simulink library "outp"  (R2021b)
(part 8 of 10)

      link override Signal_Override/_ovrdflg: Value=KOUTP_EC1EMSupVarRTSC1MSG_cnt_ovrdflg
      link override Signal_Override/_ovrdval: Value=KOUTP_EC1EMSupVarRTSC1MSG_cnt_ovrdval
  VTQD_EC1PercTorqIdleP1_pct_Inproc : FVT_lib/outp/OverrideAndLimit  SystemSampleTime=-1  VariantActivationTime=update diagram  Latency=0  AutoFrameSizeCalculation=off
      link override Signal_Limit/_maxval: Value=KOUTP_EC1PercTorqIdleP1_pct_maxval
      link override Signal_Limit/_minval: Value=KOUTP_EC1PercTorqIdleP1_pct_minval
      link override Signal_Override/_ovrdflg: Value=KOUTP_EC1PercTorqIdleP1_pct_ovrdflg
      link override Signal_Override/_ovrdval: Value=KOUTP_EC1PercTorqIdleP1_pct_ovrdval
  VTQD_EC1PercTorqIdleP2_pct_Inproc : FVT_lib/outp/OverrideAndLimit  SystemSampleTime=-1  VariantActivationTime=update diagram  Latency=0  AutoFrameSizeCalculation=off
      link override Signal_Limit/_maxval: Value=KOUTP_EC1PercTorqIdleP2_pct_maxval
      link override Signal_Limit/_minval: Value=KOUTP_EC1PercTorqIdleP2_pct_minval
      link override Signal_Override/_ovrdflg: Value=KOUTP_EC1PercTorqIdleP2_pct_ovrdflg
      link override Signal_Override/_ovrdval: Value=KOUTP_EC1PercTorqIdleP2_pct_ovrdval
  VTQD_EC1PercTorqIdleP3_pct_Inproc : FVT_lib/outp/OverrideAndLimit  SystemSampleTime=-1  VariantActivationTime=update diagram  Latency=0  AutoFrameSizeCalculation=off
      link override Signal_Limit/_maxval: Value=KOUTP_EC1PercTorqIdleP3_pct_maxval
      link override Signal_Limit/_minval: Value=KOUTP_EC1PercTorqIdleP3_pct_minval
      link override Signal_Override/_ovrdflg: Value=KOUTP_EC1PercTorqIdleP3_pct_ovrdflg
      link override Signal_Override/_ovrdval: Value=KOUTP_EC1PercTorqIdleP3_pct_ovrdval
  VTQD_EC1PercTorqIdleP4_pct_Inproc : FVT_lib/outp/OverrideAndLimit  SystemSampleTime=-1  VariantActivationTime=update diagram  Latency=0  AutoFrameSizeCalculation=off
      link override Signal_Limit/_maxval: Value=KOUTP_EC1PercTorqIdleP4_pct_maxval
      link override Signal_Limit/_minval: Value=KOUTP_EC1PercTorqIdleP4_pct_minval
      link override Signal_Override/_ovrdflg: Value=KOUTP_EC1PercTorqIdleP4_pct_ovrdflg
      link override Signal_Override/_ovrdval: Value=KOUTP_EC1PercTorqIdleP4_pct_ovrdval
  VTQD_EC1PercTorqIdleP5_pct_Inproc : FVT_lib/outp/OverrideAndLimit  SystemSampleTime=-1  VariantActivationTime=update diagram  Latency=0  AutoFrameSizeCalculation=off
      link override Signal_Limit/_maxval: Value=KOUTP_EC1PercTorqIdleP5_pct_maxval
      link override Signal_Limit/_minval: Value=KOUTP_EC1PercTorqIdleP5_pct_minval
      link override Signal_Override/_ovrdflg: Value=KOUTP_EC1PercTorqIdleP5_pct_ovrdflg
      link override Signal_Override/_ovrdval: Value=KOUTP_EC1PercTorqIdleP5_pct_ovrdval
  VTQD_EEC3EMPressLoss_pct_Inproc : FVT_lib/outp/OverrideAndLimit  SystemSampleTime=-1  VariantActivationTime=update diagram  Latency=0  AutoFrameSizeCalculation=off
      link override Signal_Limit/_maxval: Value=KOUTP_EEC3EMPressLoss_pct_maxval
      link override Signal_Limit/_minval: Value=KOUTP_EEC3EMPressLoss_pct_minval
      link override Signal_Override/_ovrdflg: Value=KOUTP_EEC3EMPressLoss_pct_ovrdflg
      link override Signal_Override/_ovrdval: Value=KOUTP_EEC3EMPressLoss_pct_ovrdval
  VTQD_EEC3NFricPercTorq_pct_Inproc : FVT_lib/outp/OverrideAndLimit  SystemSampleTime=-1  VariantActivationTime=update diagram  Latency=0  AutoFrameSizeCalculation=off
      link override Signal_Limit/_maxval: Value=KOUTP_EEC3NFricPercTorq_pct_maxval
      link override Signal_Limit/_minval: Value=KOUTP_EEC3NFricPercTorq_pct_minval
      link override Signal_Override/_ovrdflg: Value=KOUTP_EEC3NFricPercTorq_pct_ovrdflg
      link override Signal_Override/_ovrdval: Value=KOUTP_EEC3NFricPercTorq_pct_ovrdval
  VTQD_EMRC1ActEMOutSftSpd_rpm_Inproc : FVT_lib/outp/OverrideAndLimit  SystemSampleTime=-1  VariantActivationTime=update diagram  Latency=0  AutoFrameSizeCalculation=off
      link override Signal_Limit/_maxval: Value=KOUTP_EMRC1ActEMOutSftSpd_rpm_maxval
      link override Signal_Limit/_minval: Value=KOUTP_EMRC1ActEMOutSftSpd_rpm_minval
      link override Signal_Override/_ovrdflg: Value=KOUTP_EMRC1ActEMOutSftSpd_rpm_ovrdflg
      link override Signal_Override/_ovrdval: Value=KOUTP_EMRC1ActEMOutSftSpd_rpm_ovrdval
  VTQD_EMRC1ActEMpTrqHrls_pct_Inproc : FVT_lib/outp/OverrideAndLimit  SystemSampleTime=-1  VariantActivationTime=update diagram  Latency=0  AutoFrameSizeCalculation=off
      link override Signal_Limit/_maxval: Value=KOUTP_EMRC1ActEMpTrqHrls_pct_maxval
      link override Signal_Limit/_minval: Value=KOUTP_EMRC1ActEMpTrqHrls_pct_minval
      link override Signal_Override/_ovrdflg: Value=KOUTP_EMRC1ActEMpTrqHrls_pct_ovrdflg
      link override Signal_Override/_ovrdval: Value=KOUTP_EMRC1ActEMpTrqHrls_pct_ovrdval
  VTQD_EMRC1ActEMpTrq_pct_Inproc : FVT_lib/outp/OverrideAndLimit  SystemSampleTime=-1  VariantActivationTime=update diagram  Latency=0  AutoFrameSizeCalculation=off
      link override Signal_Limit/_maxval: Value=KOUTP_EMRC1ActEMpTrq_pct_maxval
      link override Signal_Limit/_minval: Value=KOUTP_EMRC1ActEMpTrq_pct_minval
      link override Signal_Override/_ovrdflg: Value=KOUTP_EMRC1ActEMpTrq_pct_ovrdflg
      link override Signal_Override/_ovrdval: Value=KOUTP_EMRC1ActEMpTrq_pct_ovrdval
  VTQD_EMRC1ActMaxAvaEMRecpTrq_pct_Inproc : FVT_lib/outp/OverrideAndLimit  SystemSampleTime=-1  VariantActivationTime=update diagram  Latency=0  AutoFrameSizeCalculation=off
      link override Signal_Limit/_maxval: Value=KOUTP_EMRC1ActMaxAvaEMRecpTrq_pct_maxval
      link override Signal_Limit/_minval: Value=KOUTP_EMRC1ActMaxAvaEMRecpTrq_pct_minval
      link override Signal_Override/_ovrdflg: Value=KOUTP_EMRC1ActMaxAvaEMRecpTrq_pct_ovrdflg
      link override Signal_Override/_ovrdval: Value=KOUTP_EMRC1ActMaxAvaEMRecpTrq_pct_ovrdval
  VTQD_EMRC1DrvDemEMRtapTrq_pct_Inproc : FVT_lib/outp/OverrideAndLimit  SystemSampleTime=-1  VariantActivationTime=update diagram  Latency=0  AutoFrameSizeCalculation=off
      link override Signal_Limit/_maxval: Value=KOUTP_EMRC1DrvDemEMRtapTrq_pct_maxval
      link override Signal_Limit/_minval: Value=KOUTP_EMRC1DrvDemEMRtapTrq_pct_minval
      link override Signal_Override/_ovrdflg: Value=KOUTP_EMRC1DrvDemEMRtapTrq_pct_ovrdflg
      link override Signal_Override/_ovrdval: Value=KOUTP_EMRC1DrvDemEMRtapTrq_pct_ovrdval
  VTQD_EMRC1EMTquModeDrvBrk_enum_Inproc : FVT_lib/outp/OverrideAndLimit  SystemSampleTime=-1  VariantActivationTime=update diagram  Latency=0  AutoFrameSizeCalculation=off
      link override Signal_Limit/_maxval: Value=KOUTP_EMRC1EMTquModeDrvBrk_enum_maxval
      link override Signal_Limit/_minval: Value=KOUTP_EMRC1EMTquModeDrvBrk_enum_minval
      link override Signal_Override/_ovrdflg: Value=KOUTP_EMRC1EMTquModeDrvBrk_enum_ovrdflg
      link override Signal_Override/_ovrdval: Value=KOUTP_EMRC1EMTquModeDrvBrk_enum_ovrdval
  VTQD_EMRC1RetSelNonEng_pct_Inproc : FVT_lib/outp/OverrideAndLimit  SystemSampleTime=-1  VariantActivationTime=update diagram  Latency=0  AutoFrameSizeCalculation=off
      link override Signal_Limit/_maxval: Value=KOUTP_EMRC1RetSelNonEng_pct_maxval
      link override Signal_Limit/_minval: Value=KOUTP_EMRC1RetSelNonEng_pct_minval
      link override Signal_Override/_ovrdflg: Value=KOUTP_EMRC1RetSelNonEng_pct_ovrdflg
      link override Signal_Override/_ovrdval: Value=KOUTP_EMRC1RetSelNonEng_pct_ovrdval
  VTQD_EMRC1SACtrlDev_cnt_Inproc : FVT_lib/outp/OverrideAndLimit  SystemSampleTime=-1  VariantActivationTime=update diagram  Latency=0  AutoFrameSizeCalculation=off
      link override Signal_Limit/_maxval: Value=KOUTP_EMRC1SACtrlDev_cnt_maxval
      link override Signal_Limit/_minval: Value=KOUTP_EMRC1SACtrlDev_cnt_minval
      link override Signal_Override/_ovrdflg: Value=KOUTP_EMRC1SACtrlDev_cnt_ovrdflg
      link override Signal_Override/_ovrdval: Value=KOUTP_EMRC1SACtrlDev_cnt_ovrdval
  VTQD_ETC1ShiftrPgs_enum_Inproc : FVT_lib/outp/OverrideAndLimit  SystemSampleTime=-1  VariantActivationTime=update diagram  Latency=0  AutoFrameSizeCalculation=off
      link override Signal_Limit/_maxval: Value=KOUTP_ETC1ShiftrPgs_enum_maxval
      link override Signal_Limit/_minval: Value=KOUTP_ETC1ShiftrPgs_enum_minval
      link override Signal_Override/_ovrdflg: Value=KOUTP_ETC1ShiftrPgs_enum_ovrdflg
      link override Signal_Override/_ovrdval: Value=KOUTP_ETC1ShiftrPgs_enum_ovrdval
  VTQD_ETC2ActDriveDirect_enum_Inproc : FVT_lib/outp/OverrideAndLimit  SystemSampleTime=-1  VariantActivationTime=update diagram  Latency=0  AutoFrameSizeCalculation=off
      link override Signal_Limit/_maxval: Value=KOUTP_ETC2ActDriveDirect_enum_maxval
      link override Signal_Limit/_minval: Value=KOUTP_ETC2ActDriveDirect_enum_minval
      link override Signal_Override/_ovrdflg: Value=KOUTP_ETC2ActDriveDirect_enum_ovrdflg
      link override Signal_Override/_ovrdval: Value=KOUTP_ETC2ActDriveDirect_enum_ovrdval
  VTQD_EVCU1ActDrvMode_enum_Inproc : FVT_lib/outp/OverrideAndLimit  SystemSampleTime=-1  VariantActivationTime=update diagram  Latency=0  AutoFrameSizeCalculation=off
      link override Signal_Limit/_maxval: Value=KOUTP_EVCU1ActDrvMode_enum_maxval
      link override Signal_Limit/_minval: Value=KOUTP_EVCU1ActDrvMode_enum_minval
      link override Signal_Override/_ovrdflg: Value=KOUTP_EVCU1ActDrvMode_enum_ovrdflg
      link override Signal_Override/_ovrdval: Value=KOUTP_EVCU1ActDrvMode_enum_ovrdval
  VTQD_EVCU1EBrakeTorqLow_enum_Inproc : FVT_lib/outp/OverrideAndLimit  SystemSampleTime=-1  VariantActivationTime=update diagram  Latency=0  AutoFrameSizeCalculation=off
      link override Signal_Limit/_maxval: Value=KOUTP_EVCU1EBrakeTorqLow_enum_maxval
      link override Signal_Limit/_minval: Value=KOUTP_EVCU1EBrakeTorqLow_enum_minval
      link override Signal_Override/_ovrdflg: Value=KOUTP_EVCU1EBrakeTorqLow_enum_ovrdflg
      link override Signal_Override/_ovrdval: Value=KOUTP_EVCU1EBrakeTorqLow_enum_ovrdval
  VTQD_EVCU1EMotorOvrerSpd_enum_Inproc : FVT_lib/outp/OverrideAndLimit  SystemSampleTime=-1  VariantActivationTime=update diagram  Latency=0  AutoFrameSizeCalculation=off
      link override Signal_Limit/_maxval: Value=KOUTP_EVCU1EMotorOvrerSpd_enum_maxval
      link override Signal_Limit/_minval: Value=KOUTP_EVCU1EMotorOvrerSpd_enum_minval
      link override Signal_Override/_ovrdflg: Value=KOUTP_EVCU1EMotorOvrerSpd_enum_ovrdflg
      link override Signal_Override/_ovrdval: Value=KOUTP_EVCU1EMotorOvrerSpd_enum_ovrdval
  VTQD_EVCU1EMotorPerformance_pct_Inproc : FVT_lib/outp/OverrideAndLimit  SystemSampleTime=-1  VariantActivationTime=update diagram  Latency=0  AutoFrameSizeCalculation=off
      link override Signal_Limit/_maxval: Value=KOUTP_EVCU1EMotorPerformance_pct_maxval
      link override Signal_Limit/_minval: Value=KOUTP_EVCU1EMotorPerformance_pct_minval
      link override Signal_Override/_ovrdflg: Value=KOUTP_EVCU1EMotorPerformance_pct_ovrdflg
      link override Signal_Override/_ovrdval: Value=KOUTP_EVCU1EMotorPerformance_pct_ovrdval
  VTQD_EVCU1EMotorSpd_rpm_Inproc : FVT_lib/outp/OverrideAndLimit  SystemSampleTime=-1  VariantActivationTime=update diagram  Latency=0  AutoFrameSizeCalculation=off
      link override Signal_Limit/_maxval: Value=KOUTP_EVCU1EMotorSpd_rpm_maxval
      link override Signal_Limit/_minval: Value=KOUTP_EVCU1EMotorSpd_rpm_minval
      link override Signal_Override/_ovrdflg: Value=KOUTP_EVCU1EMotorSpd_rpm_ovrdflg
      link override Signal_Override/_ovrdval: Value=KOUTP_EVCU1EMotorSpd_rpm_ovrdval
  VTQD_EVCU1RecuperHighSta_enum_Inproc : FVT_lib/outp/OverrideAndLimit  SystemSampleTime=-1  VariantActivationTime=update diagram  Latency=0  AutoFrameSizeCalculation=off
      link override Signal_Limit/_maxval: Value=KOUTP_EVCU1RecuperHighSta_enum_maxval
      link override Signal_Limit/_minval: Value=KOUTP_EVCU1RecuperHighSta_enum_minval
      link override Signal_Override/_ovrdflg: Value=KOUTP_EVCU1RecuperHighSta_enum_ovrdflg
      link override Signal_Override/_ovrdval: Value=KOUTP_EVCU1RecuperHighSta_enum_ovrdval
  VTQD_EVCU1WheelSlipdet_enum_Inproc : FVT_lib/outp/OverrideAndLimit  SystemSampleTime=-1  VariantActivationTime=update diagram  Latency=0  AutoFrameSizeCalculation=off
      link override Signal_Limit/_maxval: Value=KOUTP_EVCU1WheelSlipdet_enum_maxval
      link override Signal_Limit/_minval: Value=KOUTP_EVCU1WheelSlipdet_enum_minval
      link override Signal_Override/_ovrdflg: Value=KOUTP_EVCU1WheelSlipdet_enum_ovrdflg
      link override Signal_Override/_ovrdval: Value=KOUTP_EVCU1WheelSlipdet_enum_ovrdval
  VTQD_EVCU2MaxTorqAvail_pct_Inproc : FVT_lib/outp/OverrideAndLimit  SystemSampleTime=-1  VariantActivationTime=update diagram  Latency=0  AutoFrameSizeCalculation=off
      link override Signal_Limit/_maxval: Value=KOUTP_EVCU2MaxTorqAvail_pct_maxval
      link override Signal_Limit/_minval: Value=KOUTP_EVCU2MaxTorqAvail_pct_minval
      link override Signal_Override/_ovrdflg: Value=KOUTP_EVCU2MaxTorqAvail_pct_ovrdflg
      link override Signal_Override/_ovrdval: Value=KOUTP_EVCU2MaxTorqAvail_pct_ovrdval
  VTQD_EVCU2MinTorqAvail_pct_Inproc : FVT_lib/outp/OverrideAndLimit  SystemSampleTime=-1  VariantActivationTime=update diagram  Latency=0  AutoFrameSizeCalculation=off
      link override Signal_Limit/_maxval: Value=KOUTP_EVCU2MinTorqAvail_pct_maxval
      link override Signal_Limit/_minval: Value=KOUTP_EVCU2MinTorqAvail_pct_minval
      link override Signal_Override/_ovrdflg: Value=KOUTP_EVCU2MinTorqAvail_pct_ovrdflg
      link override Signal_Override/_ovrdval: Value=KOUTP_EVCU2MinTorqAvail_pct_ovrdval
  VTQD_GearFlashIndDis_flg_Inproc : FVT_lib/outp/OverrideAndLimit  SystemSampleTime=-1  VariantActivationTime=update diagram  Latency=0  AutoFrameSizeCalculation=off
      link override Signal_Limit/_maxval: Value=KOUTP_GearFlashIndDis_flg_maxval
      link override Signal_Limit/_minval: Value=KOUTP_GearFlashIndDis_flg_minval
      link override Signal_Override/_ovrdflg: Value=KOUTP_GearFlashIndDis_flg_ovrdflg
      link override Signal_Override/_ovrdval: Value=KOUTP_GearFlashIndDis_flg_ovrdval
  VTQD_GearFlashInd_flg_Inproc : FVT_lib/outp/OverrideAndLimit  SystemSampleTime=-1  VariantActivationTime=update diagram  Latency=0  AutoFrameSizeCalculation=off
      link override Signal_Limit/_maxval: Value=KOUTP_GearFlashInd_flg_maxval
      link override Signal_Limit/_minval: Value=KOUTP_GearFlashInd_flg_minval
      link override Signal_Override/_ovrdflg: Value=KOUTP_GearFlashInd_flg_ovrdflg
      link override Signal_Override/_ovrdval: Value=KOUTP_GearFlashInd_flg_ovrdval
  VTQD_ParkingProtectWarning_flg_Inproc : FVT_lib/outp/OverrideAndLimit  SystemSampleTime=-1  VariantActivationTime=update diagram  Latency=0  AutoFrameSizeCalculation=off
      link override Signal_Limit/_maxval: Value=KOUTP_ParkingProtectWarning_flg_maxval
      link override Signal_Limit/_minval: Value=KOUTP_ParkingProtectWarning_flg_minval
      link override Signal_Override/_ovrdflg: Value=KOUTP_ParkingProtectWarning_flg_ovrdflg
      link override Signal_Override/_ovrdval: Value=KOUTP_ParkingProtectWarning_flg_ovrdval
  VTQD_RC1MaxRetSpdP2_rpm_Inproc : FVT_lib/outp/OverrideAndLimit  SystemSampleTime=-1  VariantActivationTime=update diagram  Latency=0  AutoFrameSizeCalculation=off
      link override Signal_Limit/_maxval: Value=KOUTP_RC1MaxRetSpdP2_rpm_maxval
      link override Signal_Limit/_minval: Value=KOUTP_RC1MaxRetSpdP2_rpm_minval
      link override Signal_Override/_ovrdflg: Value=KOUTP_RC1MaxRetSpdP2_rpm_ovrdflg
      link override Signal_Override/_ovrdval: Value=KOUTP_RC1MaxRetSpdP2_rpm_ovrdval
  VTQD_RC1MaxRetSpdP3_rpm_Inproc : FVT_lib/outp/OverrideAndLimit  SystemSampleTime=-1  VariantActivationTime=update diagram  Latency=0  AutoFrameSizeCalculation=off
      link override Signal_Limit/_maxval: Value=KOUTP_RC1MaxRetSpdP3_rpm_maxval
      link override Signal_Limit/_minval: Value=KOUTP_RC1MaxRetSpdP3_rpm_minval
      link override Signal_Override/_ovrdflg: Value=KOUTP_RC1MaxRetSpdP3_rpm_ovrdflg
      link override Signal_Override/_ovrdval: Value=KOUTP_RC1MaxRetSpdP3_rpm_ovrdval
  VTQD_RC1PctTrqIdleP1_pct_Inproc : FVT_lib/outp/OverrideAndLimit  SystemSampleTime=-1  VariantActivationTime=update diagram  Latency=0  AutoFrameSizeCalculation=off
      link override Signal_Limit/_maxval: Value=KOUTP_RC1PctTrqIdleP1_pct_maxval
      link override Signal_Limit/_minval: Value=KOUTP_RC1PctTrqIdleP1_pct_minval
      link override Signal_Override/_ovrdflg: Value=KOUTP_RC1PctTrqIdleP1_pct_ovrdflg
      link override Signal_Override/_ovrdval: Value=KOUTP_RC1PctTrqIdleP1_pct_ovrdval
  VTQD_RC1PctTrqP3_pct_Inproc : FVT_lib/outp/OverrideAndLimit  SystemSampleTime=-1  VariantActivationTime=update diagram  Latency=0  AutoFrameSizeCalculation=off
      link override Signal_Limit/_maxval: Value=KOUTP_RC1PctTrqP3_pct_maxval
      link override Signal_Limit/_minval: Value=KOUTP_RC1PctTrqP3_pct_minval
      link override Signal_Override/_ovrdflg: Value=KOUTP_RC1PctTrqP3_pct_ovrdflg
      link override Signal_Override/_ovrdval: Value=KOUTP_RC1PctTrqP3_pct_ovrdval
  VTQD_RC1PctTrqP4_pct_Inproc : FVT_lib/outp/OverrideAndLimit  SystemSampleTime=-1  VariantActivationTime=update diagram  Latency=0  AutoFrameSizeCalculation=off
      link override Signal_Limit/_maxval: Value=KOUTP_RC1PctTrqP4_pct_maxval
      link override Signal_Limit/_minval: Value=KOUTP_RC1PctTrqP4_pct_minval
      link override Signal_Override/_ovrdflg: Value=KOUTP_RC1PctTrqP4_pct_ovrdflg
      link override Signal_Override/_ovrdval: Value=KOUTP_RC1PctTrqP4_pct_ovrdval
  VTQD_RC1PctTrqPekTrqP5_pct_Inproc : FVT_lib/outp/OverrideAndLimit  SystemSampleTime=-1  VariantActivationTime=update diagram  Latency=0  AutoFrameSizeCalculation=off
      link override Signal_Limit/_maxval: Value=KOUTP_RC1PctTrqPekTrqP5_pct_maxval
      link override Signal_Limit/_minval: Value=KOUTP_RC1PctTrqPekTrqP5_pct_minval
      link override Signal_Override/_ovrdflg: Value=KOUTP_RC1PctTrqPekTrqP5_pct_ovrdflg
      link override Signal_Override/_ovrdval: Value=KOUTP_RC1PctTrqPekTrqP5_pct_ovrdval
  VTQD_RC1RefRetTrq_Nm_Inproc : FVT_lib/outp/OverrideAndLimit  SystemSampleTime=-1  VariantActivationTime=update diagram  Latency=0  AutoFrameSizeCalculation=off
      link override Signal_Limit/_maxval: Value=KOUTP_RC1RefRetTrq_Nm_maxval
      link override Signal_Limit/_minval: Value=KOUTP_RC1RefRetTrq_Nm_minval
      link override Signal_Override/_ovrdflg: Value=KOUTP_RC1RefRetTrq_Nm_ovrdflg
      link override Signal_Override/_ovrdval: Value=KOUTP_RC1RefRetTrq_Nm_ovrdval
  VTQD_RC1RetCtrlMth_enum_Inproc : FVT_lib/outp/OverrideAndLimit  SystemSampleTime=-1  VariantActivationTime=update diagram  Latency=0  AutoFrameSizeCalculation=off
      link override Signal_Limit/_maxval: Value=KOUTP_RC1RetCtrlMth_enum_maxval
      link override Signal_Limit/_minval: Value=KOUTP_RC1RetCtrlMth_enum_minval
      link override Signal_Override/_ovrdflg: Value=KOUTP_RC1RetCtrlMth_enum_ovrdflg
      link override Signal_Override/_ovrdval: Value=KOUTP_RC1RetCtrlMth_enum_ovrdval
  VTQD_RC1RetLocat_enum_Inproc : FVT_lib/outp/OverrideAndLimit  SystemSampleTime=-1  VariantActivationTime=update diagram  Latency=0  AutoFrameSizeCalculation=off
      link override Signal_Limit/_maxval: Value=KOUTP_RC1RetLocat_enum_maxval
      link override Signal_Limit/_minval: Value=KOUTP_RC1RetLocat_enum_minval
      link override Signal_Override/_ovrdflg: Value=KOUTP_RC1RetLocat_enum_ovrdflg
      link override Signal_Override/_ovrdval: Value=KOUTP_RC1RetLocat_enum_ovrdval
  VTQD_RC1RetSpdIdleP1_rpm_Inproc : FVT_lib/outp/OverrideAndLimit  SystemSampleTime=-1  VariantActivationTime=update diagram  Latency=0  AutoFrameSizeCalculation=off
      link override Signal_Limit/_maxval: Value=KOUTP_RC1RetSpdIdleP1_rpm_maxval
      link override Signal_Limit/_minval: Value=KOUTP_RC1RetSpdIdleP1_rpm_minval
      link override Signal_Override/_ovrdflg: Value=KOUTP_RC1RetSpdIdleP1_rpm_ovrdflg
      link override Signal_Override/_ovrdval: Value=KOUTP_RC1RetSpdIdleP1_rpm_ovrdval
  VTQD_RC1RetSpdP2_pct_Inproc : FVT_lib/outp/OverrideAndLimit  SystemSampleTime=-1  VariantActivationTime=update diagram  Latency=0  AutoFrameSizeCalculation=off
      link override Signal_Limit/_maxval: Value=KOUTP_RC1RetSpdP2_pct_maxval
      link override Signal_Limit/_minval: Value=KOUTP_RC1RetSpdP2_pct_minval
      link override Signal_Override/_ovrdflg: Value=KOUTP_RC1RetSpdP2_pct_ovrdflg
      link override Signal_Override/_ovrdval: Value=KOUTP_RC1RetSpdP2_pct_ovrdval
  VTQD_RC1RetSpdP4_rpm_Inproc : FVT_lib/outp/OverrideAndLimit  SystemSampleTime=-1  VariantActivationTime=update diagram  Latency=0  AutoFrameSizeCalculation=off
      link override Signal_Limit/_maxval: Value=KOUTP_RC1RetSpdP4_rpm_maxval
      link override Signal_Limit/_minval: Value=KOUTP_RC1RetSpdP4_rpm_minval
      link override Signal_Override/_ovrdflg: Value=KOUTP_RC1RetSpdP4_rpm_ovrdflg
      link override Signal_Override/_ovrdval: Value=KOUTP_RC1RetSpdP4_rpm_ovrdval
  VTQD_RC1RetSpdPekTrqP5_Nm_Inproc : FVT_lib/outp/OverrideAndLimit  SystemSampleTime=-1  VariantActivationTime=update diagram  Latency=0  AutoFrameSizeCalculation=off
      link override Signal_Limit/_maxval: Value=KOUTP_RC1RetSpdPekTrqP5_Nm_maxval
      link override Signal_Limit/_minval: Value=KOUTP_RC1RetSpdPekTrqP5_Nm_minval
      link override Signal_Override/_ovrdflg: Value=KOUTP_RC1RetSpdPekTrqP5_Nm_ovrdflg
      link override Signal_Override/_ovrdval: Value=KOUTP_RC1RetSpdPekTrqP5_Nm_ovrdval
  VTQD_RC1RetType_enum_Inproc : FVT_lib/outp/OverrideAndLimit  SystemSampleTime=-1  VariantActivationTime=update diagram  Latency=0  AutoFrameSizeCalculation=off
      link override Signal_Limit/_maxval: Value=KOUTP_RC1RetType_enum_maxval
      link override Signal_Limit/_minval: Value=KOUTP_RC1RetType_enum_minval
      link override Signal_Override/_ovrdflg: Value=KOUTP_RC1RetType_enum_ovrdflg
      link override Signal_Override/_ovrdval: Value=KOUTP_RC1RetType_enum_ovrdval
  VTQD_SpdLimSta_flg_Inproc : FVT_lib/outp/OverrideAndLimit  SystemSampleTime=-1  VariantActivationTime=update diagram  Latency=0  AutoFrameSizeCalculation=off
      link override Signal_Limit/_maxval: Value=KOUTP_SpdLimSta_flg_maxval
      link override Signal_Limit/_minval: Value=KOUTP_SpdLimSta_flg_minval
      link override Signal_Override/_ovrdflg: Value=KOUTP_SpdLimSta_flg_ovrdflg
      link override Signal_Override/_ovrdval: Value=KOUTP_SpdLimSta_flg_ovrdval
  VTQD_TMTqReq_Nm_Inproc : FVT_lib/outp/OverrideAndLimit  SystemSampleTime=-1  VariantActivationTime=update diagram  Latency=0  AutoFrameSizeCalculation=off
      link override Signal_Limit/_maxval: Value=KOUTP_TMTqReq_Nm_maxval
      link override Signal_Limit/_minval: Value=KOUTP_TMTqReq_Nm_minval
      link override Signal_Override/_ovrdflg: Value=KOUTP_TMTqReq_Nm_ovrdflg
      link override Signal_Override/_ovrdval: Value=KOUTP_TMTqReq_Nm_ovrdval
  VTQD_TUpAIND_enum_Inproc : FVT_lib/outp/OverrideAndLimit  SystemSampleTime=-1  VariantActivationTime=update diagram  Latency=0  AutoFrameSizeCalculation=off
      link override Signal_Limit/_maxval: Value=KOUTP_TUpAIND_enum_maxval
      link override Signal_Limit/_minval: Value=KOUTP_TUpAIND_enum_minval
      link override Signal_Override/_ovrdflg: Value=KOUTP_TUpAIND_enum_ovrdflg
      link override Signal_Override/_ovrdval: Value=KOUTP_TUpAIND_enum_ovrdval
  VTQD_VCU4PweLmtInd_flg_Inproc : FVT_lib/outp/OverrideAndLimit  SystemSampleTime=-1  VariantActivationTime=update diagram  Latency=0  AutoFrameSizeCalculation=off
      link override Signal_Limit/_maxval: Value=KOUTP_VCU4PweLmtInd_flg_maxval
      link override Signal_Limit/_minval: Value=KOUTP_VCU4PweLmtInd_flg_minval
      link override Signal_Override/_ovrdflg: Value=KOUTP_VCU4PweLmtInd_flg_ovrdflg
      link override Signal_Override/_ovrdval: Value=KOUTP_VCU4PweLmtInd_flg_ovrdval
  VTQD_VCUBCMBuzzReq_flg_Inproc : FVT_lib/outp/OverrideAndLimit  SystemSampleTime=-1  VariantActivationTime=update diagram  Latency=0  AutoFrameSizeCalculation=off
      link override Signal_Limit/_maxval: Value=KOUTP_VCUBCMBuzzReq_flg_maxval
      link override Signal_Limit/_minval: Value=KOUTP_VCUBCMBuzzReq_flg_minval
      link override Signal_Override/_ovrdflg: Value=KOUTP_VCUBCMBuzzReq_flg_ovrdflg
      link override Signal_Override/_ovrdval: Value=KOUTP_VCUBCMBuzzReq_flg_ovrdval
  VTQD_VCUEBSHBSw_enum_Inproc : FVT_lib/outp/OverrideAndLimit  SystemSampleTime=-1  VariantActivationTime=update diagram  Latency=0  AutoFrameSizeCalculation=off
      link override Signal_Limit/_maxval: Value=KOUTP_VCUEBSHBSw_enum_maxval
      link override Signal_Limit/_minval: Value=KOUTP_VCUEBSHBSw_enum_minval
      link override Signal_Override/_ovrdflg: Value=KOUTP_VCUEBSHBSw_enum_ovrdflg
      link override Signal_Override/_ovrdval: Value=KOUTP_VCUEBSHBSw_enum_ovrdval
  VTQD_VCUEBSHHSw_enum_Inproc : FVT_lib/outp/OverrideAndLimit  SystemSampleTime=-1  VariantActivationTime=update diagram  Latency=0  AutoFrameSizeCalculation=off
      link override Signal_Limit/_maxval: Value=KOUTP_VCUEBSHHSw_enum_maxval
      link override Signal_Limit/_minval: Value=KOUTP_VCUEBSHHSw_enum_minval
      link override Signal_Override/_ovrdflg: Value=KOUTP_VCUEBSHHSw_enum_ovrdflg
      link override Signal_Override/_ovrdval: Value=KOUTP_VCUEBSHHSw_enum_ovrdval
  VTQD_VCUEBSRd4BR_enum_Inproc : FVT_lib/outp/OverrideAndLimit  SystemSampleTime=-1  VariantActivationTime=update diagram  Latency=0  AutoFrameSizeCalculation=off
      link override Signal_Limit/_maxval: Value=KOUTP_VCUEBSRd4BR_enum_maxval
      link override Signal_Limit/_minval: Value=KOUTP_VCUEBSRd4BR_enum_minval
      link override Signal_Override/_ovrdflg: Value=KOUTP_VCUEBSRd4BR_enum_ovrdflg
      link override Signal_Override/_ovrdval: Value=KOUTP_VCUEBSRd4BR_enum_ovrdval
  VTQD_VCUMCUCtrlMdTQD_enum_Inproc : FVT_lib/outp/OverrideAndLimit  SystemSampleTime=-1  VariantActivationTime=update diagram  Latency=0  AutoFrameSizeCalculation=off
      link override Signal_Limit/_maxval: Value=KOUTP_VCUMCUCtrlMdTQD_enum_maxval
      link override Signal_Limit/_minval: Value=KOUTP_VCUMCUCtrlMdTQD_enum_minval
      link override Signal_Override/_ovrdflg: Value=KOUTP_VCUMCUCtrlMdTQD_enum_ovrdflg
      link override Signal_Override/_ovrdval: Value=KOUTP_VCUMCUCtrlMdTQD_enum_ovrdval
  VTQD_VCUMCUDemHiPosVal_rpm_Inproc : FVT_lib/outp/OverrideAndLimit  SystemSampleTime=-1  VariantActivationTime=update diagram  Latency=0  AutoFrameSizeCalculation=off
      link override Signal_Limit/_maxval: Value=KOUTP_VCUMCUDemHiPosVal_rpm_maxval
      link override Signal_Limit/_minval: Value=KOUTP_VCUMCUDemHiPosVal_rpm_minval
      link override Signal_Override/_ovrdflg: Value=KOUTP_VCUMCUDemHiPosVal_rpm_ovrdflg
      link override Signal_Override/_ovrdval: Value=KOUTP_VCUMCUDemHiPosVal_rpm_ovrdval
  VTQD_VCUMCUDemLoNegVal_rpm_Inproc : FVT_lib/outp/OverrideAndLimit  SystemSampleTime=-1  VariantActivationTime=update diagram  Latency=0  AutoFrameSizeCalculation=off
      link override Signal_Limit/_maxval: Value=KOUTP_VCUMCUDemLoNegVal_rpm_maxval
      link override Signal_Limit/_minval: Value=KOUTP_VCUMCUDemLoNegVal_rpm_minval
      link override Signal_Override/_ovrdflg: Value=KOUTP_VCUMCUDemLoNegVal_rpm_ovrdflg
      link override Signal_Override/_ovrdval: Value=KOUTP_VCUMCUDemLoNegVal_rpm_ovrdval
  VTQD_VCUMCUDemSpd_rpm_Inproc : FVT_lib/outp/OverrideAndLimit  SystemSampleTime=-1  VariantActivationTime=update diagram  Latency=0  AutoFrameSizeCalculation=off
      link override Signal_Limit/_maxval: Value=KOUTP_VCUMCUDemSpd_rpm_maxval
      link override Signal_Limit/_minval: Value=KOUTP_VCUMCUDemSpd_rpm_minval
      link override Signal_Override/_ovrdflg: Value=KOUTP_VCUMCUDemSpd_rpm_ovrdflg
      link override Signal_Override/_ovrdval: Value=KOUTP_VCUMCUDemSpd_rpm_ovrdval
  VTQD_VCUMCUFootBrk_flg_Inproc : FVT_lib/outp/OverrideAndLimit  SystemSampleTime=-1  VariantActivationTime=update diagram  Latency=0  AutoFrameSizeCalculation=off
      link override Signal_Limit/_maxval: Value=KOUTP_VCUMCUFootBrk_flg_maxval
      link override Signal_Limit/_minval: Value=KOUTP_VCUMCUFootBrk_flg_minval
      link override Signal_Override/_ovrdflg: Value=KOUTP_VCUMCUFootBrk_flg_ovrdflg
      link override Signal_Override/_ovrdval: Value=KOUTP_VCUMCUFootBrk_flg_ovrdval
  VTQD_VCUMCUGearSta_enum_Inproc : FVT_lib/outp/OverrideAndLimit  SystemSampleTime=-1  VariantActivationTime=update diagram  Latency=0  AutoFrameSizeCalculation=off
      link override Signal_Limit/_maxval: Value=KOUTP_VCUMCUGearSta_enum_maxval
      link override Signal_Limit/_minval: Value=KOUTP_VCUMCUGearSta_enum_minval
      link override Signal_Override/_ovrdflg: Value=KOUTP_VCUMCUGearSta_enum_ovrdflg
      link override Signal_Override/_ovrdval: Value=KOUTP_VCUMCUGearSta_enum_ovrdval
  VTQD_VCUMCUHandBrk_flg_Inproc : FVT_lib/outp/OverrideAndLimit  SystemSampleTime=-1  VariantActivationTime=update diagram  Latency=0  AutoFrameSizeCalculation=off
      link override Signal_Limit/_maxval: Value=KOUTP_VCUMCUHandBrk_flg_maxval
      link override Signal_Limit/_minval: Value=KOUTP_VCUMCUHandBrk_flg_minval
      link override Signal_Override/_ovrdflg: Value=KOUTP_VCUMCUHandBrk_flg_ovrdflg
      link override Signal_Override/_ovrdval: Value=KOUTP_VCUMCUHandBrk_flg_ovrdval
  VTQD_VCUTMVehSpd_kph_Inproc : FVT_lib/outp/OverrideAndLimit  SystemSampleTime=-1  VariantActivationTime=update diagram  Latency=0  AutoFrameSizeCalculation=off
      link override Signal_Limit/_maxval: Value=KOUTP_VCUTMVehSpd_kph_maxval
      link override Signal_Limit/_minval: Value=KOUTP_VCUTMVehSpd_kph_minval
      link override Signal_Override/_ovrdflg: Value=KOUTP_VCUTMVehSpd_kph_ovrdflg
      link override Signal_Override/_ovrdval: Value=KOUTP_VCUTMVehSpd_kph_ovrdval
  VTQD_VehAcclLimitTG_mps2_Inproc : FVT_lib/outp/OverrideAndLimit  SystemSampleTime=-1  VariantActivationTime=update diagram  Latency=0  AutoFrameSizeCalculation=off
      link override Signal_Limit/_maxval: Value=KOUTP_VehAcclLimitTG_mps2_maxval
      link override Signal_Limit/_minval: Value=KOUTP_VehAcclLimitTG_mps2_minval
      link override Signal_Override/_ovrdflg: Value=KOUTP_VehAcclLimitTG_mps2_ovrdflg
      link override Signal_Override/_ovrdval: Value=KOUTP_VehAcclLimitTG_mps2_ovrdval
  VTQD_VehSpdLimitTG_kph_Inproc : FVT_lib/outp/OverrideAndLimit  SystemSampleTime=-1  VariantActivationTime=update diagram  Latency=0  AutoFrameSizeCalculation=off
      link override Signal_Limit/_maxval: Value=KOUTP_VehSpdLimitTG_kph_maxval
      link override Signal_Limit/_minval: Value=KOUTP_VehSpdLimitTG_kph_minval
      link override Signal_Override/_ovrdflg: Value=KOUTP_VehSpdLimitTG_kph_ovrdflg
      link override Signal_Override/_ovrdval: Value=KOUTP_VehSpdLimitTG_kph_ovrdval
  VTQR_FrTMTqReq_Nm_Inproc : FVT_lib/outp/OverrideAndLimit  SystemSampleTime=-1  VariantActivationTime=update diagram  Latency=0  AutoFrameSizeCalculation=off
      link override Signal_Limit/_maxval: Value=KOUTP_FrTMTqReq_Nm_maxval
      link override Signal_Limit/_minval: Value=KOUTP_FrTMTqReq_Nm_minval
      link override Signal_Override/_ovrdflg: Value=KOUTP_FrTMTqReq_Nm_ovrdflg
      link override Signal_Override/_ovrdval: Value=KOUTP_FrTMTqReq_Nm_ovrdval
  VTQR_RrTMTqReq_Nm_Inproc : FVT_lib/outp/OverrideAndLimit  SystemSampleTime=-1  VariantActivationTime=update diagram  Latency=0  AutoFrameSizeCalculation=off
      link override Signal_Limit/_maxval: Value=KOUTP_RrTMTqReq_Nm_maxval
      link override Signal_Limit/_minval: Value=KOUTP_RrTMTqReq_Nm_minval
      link override Signal_Override/_ovrdflg: Value=KOUTP_RrTMTqReq_Nm_ovrdflg
      link override Signal_Override/_ovrdval: Value=KOUTP_RrTMTqReq_Nm_ovrdval
  VV2L_HVPO120VGrpALDSt_enum_Inproc : FVT_lib/outp/OverrideAndLimit  SystemSampleTime=-1  VariantActivationTime=update diagram  Latency=0  AutoFrameSizeCalculation=off
      link override Signal_Limit/_maxval: Value=KOUTP_HVPO120VGrpALDSt_enum_maxval
      link override Signal_Limit/_minval: Value=KOUTP_HVPO120VGrpALDSt_enum_minval
      link override Signal_Override/_ovrdflg: Value=KOUTP_HVPO120VGrpALDSt_enum_ovrdflg
      link override Signal_Override/_ovrdval: Value=KOUTP_HVPO120VGrpALDSt_enum_ovrdval
  VV2L_HVPO120VGrpBLDSt_enum_Inproc : FVT_lib/outp/OverrideAndLimit  SystemSampleTime=-1  VariantActivationTime=update diagram  Latency=0  AutoFrameSizeCalculation=off
      link override Signal_Limit/_maxval: Value=KOUTP_HVPO120VGrpBLDSt_enum_maxval
      link override Signal_Limit/_minval: Value=KOUTP_HVPO120VGrpBLDSt_enum_minval
      link override Signal_Override/_ovrdflg: Value=KOUTP_HVPO120VGrpBLDSt_enum_ovrdflg
      link override Signal_Override/_ovrdval: Value=KOUTP_HVPO120VGrpBLDSt_enum_ovrdval
  VV2L_ReqOBCExtrV2LEna_enum_Inproc : FVT_lib/outp/OverrideAndLimit  SystemSampleTime=-1  VariantActivationTime=update diagram  Latency=0  AutoFrameSizeCalculation=off
      link override Signal_Limit/_maxval: Value=KOUTP_ReqOBCExtrV2LEna_enum_maxval
      link override Signal_Limit/_minval: Value=KOUTP_ReqOBCExtrV2LEna_enum_minval
      link override Signal_Override/_ovrdflg: Value=KOUTP_ReqOBCExtrV2LEna_enum_ovrdflg
      link override Signal_Override/_ovrdval: Value=KOUTP_ReqOBCExtrV2LEna_enum_ovrdval
  VV2L_ReqOBCIntrV2LEna_enum_Inproc : FVT_lib/outp/OverrideAndLimit  SystemSampleTime=-1  VariantActivationTime=update diagram  Latency=0  AutoFrameSizeCalculation=off
      link override Signal_Limit/_maxval: Value=KOUTP_ReqOBCIntrV2LEna_enum_maxval
      link override Signal_Limit/_minval: Value=KOUTP_ReqOBCIntrV2LEna_enum_minval
      link override Signal_Override/_ovrdflg: Value=KOUTP_ReqOBCIntrV2LEna_enum_ovrdflg
      link override Signal_Override/_ovrdval: Value=KOUTP_ReqOBCIntrV2LEna_enum_ovrdval
  VV2L_ReqOBCV2LEna_enum_Inproc : FVT_lib/outp/OverrideAndLimit  SystemSampleTime=-1  VariantActivationTime=update diagram  Latency=0  AutoFrameSizeCalculation=off
      link override Signal_Limit/_maxval: Value=KOUTP_ReqOBCV2LEna_enum_maxval
      link override Signal_Limit/_minval: Value=KOUTP_ReqOBCV2LEna_enum_minval
      link override Signal_Override/_ovrdflg: Value=KOUTP_ReqOBCV2LEna_enum_ovrdflg
      link override Signal_Override/_ovrdval: Value=KOUTP_ReqOBCV2LEna_enum_ovrdval
  VV2L_ReqV2LIVIDisChrg_enum_Inproc : FVT_lib/outp/OverrideAndLimit  SystemSampleTime=-1  VariantActivationTime=update diagram  Latency=0  AutoFrameSizeCalculation=off
      link override Signal_Limit/_maxval: Value=KOUTP_ReqV2LIVIDisChrg_enum_maxval
      link override Signal_Limit/_minval: Value=KOUTP_ReqV2LIVIDisChrg_enum_minval
      link override Signal_Override/_ovrdflg: Value=KOUTP_ReqV2LIVIDisChrg_enum_ovrdflg
      link override Signal_Override/_ovrdval: Value=KOUTP_ReqV2LIVIDisChrg_enum_ovrdval
  VV2L_ReqV2LIVIPopup_enum_Inproc : FVT_lib/outp/OverrideAndLimit  SystemSampleTime=-1  VariantActivationTime=update diagram  Latency=0  AutoFrameSizeCalculation=off
      link override Signal_Limit/_maxval: Value=KOUTP_ReqV2LIVIPopup_enum_maxval
      link override Signal_Limit/_minval: Value=KOUTP_ReqV2LIVIPopup_enum_minval
      link override Signal_Override/_ovrdflg: Value=KOUTP_ReqV2LIVIPopup_enum_ovrdflg
      link override Signal_Override/_ovrdval: Value=KOUTP_ReqV2LIVIPopup_enum_ovrdval
  VVMC_ACCComfortBandLower_mps2_Inproc : FVT_lib/outp/OverrideAndLimit  SystemSampleTime=-1  VariantActivationTime=update diagram  Latency=0  AutoFrameSizeCalculation=off
      link override Signal_Limit/_maxval: Value=KOUTP_ACCComfortBandLower_mps2_maxval
      link override Signal_Limit/_minval: Value=KOUTP_ACCComfortBandLower_mps2_minval
      link override Signal_Override/_ovrdflg: Value=KOUTP_ACCComfortBandLower_mps2_ovrdflg
      link override Signal_Override/_ovrdval: Value=KOUTP_ACCComfortBandLower_mps2_ovrdval
  VVMC_ACCComfortBandUpper_mps2_Inproc : FVT_lib/outp/OverrideAndLimit  SystemSampleTime=-1  VariantActivationTime=update diagram  Latency=0  AutoFrameSizeCalculation=off
      link override Signal_Limit/_maxval: Value=KOUTP_ACCComfortBandUpper_mps2_maxval
      link override Signal_Limit/_minval: Value=KOUTP_ACCComfortBandUpper_mps2_minval
      link override Signal_Override/_ovrdflg: Value=KOUTP_ACCComfortBandUpper_mps2_ovrdflg
      link override Signal_Override/_ovrdval: Value=KOUTP_ACCComfortBandUpper_mps2_ovrdval
  VVMC_ACCCtrlAvail_flg_Inproc : FVT_lib/outp/OverrideAndLimit  SystemSampleTime=-1  VariantActivationTime=update diagram  Latency=0  AutoFrameSizeCalculation=off
      link override Signal_Limit/_maxval: Value=KOUTP_ACCCtrlAvail_flg_maxval
      link override Signal_Limit/_minval: Value=KOUTP_ACCCtrlAvail_flg_minval
      link override Signal_Override/_ovrdflg: Value=KOUTP_ACCCtrlAvail_flg_ovrdflg
      link override Signal_Override/_ovrdval: Value=KOUTP_ACCCtrlAvail_flg_ovrdval
  VVMC_ACCJerkLowerLimit_mps3_Inproc : FVT_lib/outp/OverrideAndLimit  SystemSampleTime=-1  VariantActivationTime=update diagram  Latency=0  AutoFrameSizeCalculation=off
      link override Signal_Limit/_maxval: Value=KOUTP_ACCJerkLowerLimit_mps3_maxval
      link override Signal_Limit/_minval: Value=KOUTP_ACCJerkLowerLimit_mps3_minval
      link override Signal_Override/_ovrdflg: Value=KOUTP_ACCJerkLowerLimit_mps3_ovrdflg
      link override Signal_Override/_ovrdval: Value=KOUTP_ACCJerkLowerLimit_mps3_ovrdval
  VVMC_ACCJerkUpperLimit_mps3_Inproc : FVT_lib/outp/OverrideAndLimit  SystemSampleTime=-1  VariantActivationTime=update diagram  Latency=0  AutoFrameSizeCalculation=off
      link override Signal_Limit/_maxval: Value=KOUTP_ACCJerkUpperLimit_mps3_maxval
      link override Signal_Limit/_minval: Value=KOUTP_ACCJerkUpperLimit_mps3_minval
      link override Signal_Override/_ovrdflg: Value=KOUTP_ACCJerkUpperLimit_mps3_ovrdflg
      link override Signal_Override/_ovrdval: Value=KOUTP_ACCJerkUpperLimit_mps3_ovrdval
  VVMC_ACCObjDist_m_Inproc : FVT_lib/outp/OverrideAndLimit  SystemSampleTime=-1  VariantActivationTime=update diagram  Latency=0  AutoFrameSizeCalculation=off
      link override Signal_Limit/_maxval: Value=KOUTP_ACCObjDist_m_maxval
      link override Signal_Limit/_minval: Value=KOUTP_ACCObjDist_m_minval
      link override Signal_Override/_ovrdflg: Value=KOUTP_ACCObjDist_m_ovrdflg
      link override Signal_Override/_ovrdval: Value=KOUTP_ACCObjDist_m_ovrdval
  VVMC_ACCObjDstLvl_enum_Inproc : FVT_lib/outp/OverrideAndLimit  SystemSampleTime=-1  VariantActivationTime=update diagram  Latency=0  AutoFrameSizeCalculation=off
      link override Signal_Limit/_maxval: Value=KOUTP_ACCObjDstLvl_enum_maxval
      link override Signal_Limit/_minval: Value=KOUTP_ACCObjDstLvl_enum_minval
      link override Signal_Override/_ovrdflg: Value=KOUTP_ACCObjDstLvl_enum_ovrdflg
      link override Signal_Override/_ovrdval: Value=KOUTP_ACCObjDstLvl_enum_ovrdval
  VVMC_ACCObjRelSpd_mps_Inproc : FVT_lib/outp/OverrideAndLimit  SystemSampleTime=-1  VariantActivationTime=update diagram  Latency=0  AutoFrameSizeCalculation=off
      link override Signal_Limit/_maxval: Value=KOUTP_ACCObjRelSpd_mps_maxval
      link override Signal_Limit/_minval: Value=KOUTP_ACCObjRelSpd_mps_minval
      link override Signal_Override/_ovrdflg: Value=KOUTP_ACCObjRelSpd_mps_ovrdflg
      link override Signal_Override/_ovrdval: Value=KOUTP_ACCObjRelSpd_mps_ovrdval
  VVMC_ACCPedalOvrd_flg_Inproc : FVT_lib/outp/OverrideAndLimit  SystemSampleTime=-1  VariantActivationTime=update diagram  Latency=0  AutoFrameSizeCalculation=off
      link override Signal_Limit/_maxval: Value=KOUTP_ACCPedalOvrd_flg_maxval
      link override Signal_Limit/_minval: Value=KOUTP_ACCPedalOvrd_flg_minval
      link override Signal_Override/_ovrdflg: Value=KOUTP_ACCPedalOvrd_flg_ovrdflg
      link override Signal_Override/_ovrdval: Value=KOUTP_ACCPedalOvrd_flg_ovrdval
  VVMC_ACCRequiredAccel_mps2_Inproc : FVT_lib/outp/OverrideAndLimit  SystemSampleTime=-1  VariantActivationTime=update diagram  Latency=0  AutoFrameSizeCalculation=off
      link override Signal_Limit/_maxval: Value=KOUTP_ACCRequiredAccel_mps2_maxval
      link override Signal_Limit/_minval: Value=KOUTP_ACCRequiredAccel_mps2_minval
      link override Signal_Override/_ovrdflg: Value=KOUTP_ACCRequiredAccel_mps2_ovrdflg
      link override Signal_Override/_ovrdval: Value=KOUTP_ACCRequiredAccel_mps2_ovrdval
  VVMC_ACCTakeoverReq_flg_Inproc : FVT_lib/outp/OverrideAndLimit  SystemSampleTime=-1  VariantActivationTime=update diagram  Latency=0  AutoFrameSizeCalculation=off
      link override Signal_Limit/_maxval: Value=KOUTP_ACCTakeoverReq_flg_maxval
      link override Signal_Limit/_minval: Value=KOUTP_ACCTakeoverReq_flg_minval
      link override Signal_Override/_ovrdflg: Value=KOUTP_ACCTakeoverReq_flg_ovrdflg
      link override Signal_Override/_ovrdval: Value=KOUTP_ACCTakeoverReq_flg_ovrdval
  VVMC_ACCVehHoldReq_flg_Inproc : FVT_lib/outp/OverrideAndLimit  SystemSampleTime=-1  VariantActivationTime=update diagram  Latency=0  AutoFrameSizeCalculation=off
      link override Signal_Limit/_maxval: Value=KOUTP_ACCVehHoldReq_flg_maxval
      link override Signal_Limit/_minval: Value=KOUTP_ACCVehHoldReq_flg_minval
      link override Signal_Override/_ovrdflg: Value=KOUTP_ACCVehHoldReq_flg_ovrdflg
      link override Signal_Override/_ovrdval: Value=KOUTP_ACCVehHoldReq_flg_ovrdval
  VVMC_ADASACCSta_enum_Inproc : FVT_lib/outp/OverrideAndLimit  SystemSampleTime=-1  VariantActivationTime=update diagram  Latency=0  AutoFrameSizeCalculation=off
      link override Signal_Limit/_maxval: Value=KOUTP_ADASACCSta_enum_maxval
      link override Signal_Limit/_minval: Value=KOUTP_ADASACCSta_enum_minval
      link override Signal_Override/_ovrdflg: Value=KOUTP_ADASACCSta_enum_ovrdflg
      link override Signal_Override/_ovrdval: Value=KOUTP_ADASACCSta_enum_ovrdval
  VVMC_ADASAEBReq_enum_Inproc : FVT_lib/outp/OverrideAndLimit  SystemSampleTime=-1  VariantActivationTime=update diagram  Latency=0  AutoFrameSizeCalculation=off
      link override Signal_Limit/_maxval: Value=KOUTP_ADASAEBReq_enum_maxval
      link override Signal_Limit/_minval: Value=KOUTP_ADASAEBReq_enum_minval
      link override Signal_Override/_ovrdflg: Value=KOUTP_ADASAEBReq_enum_ovrdflg
      link override Signal_Override/_ovrdval: Value=KOUTP_ADASAEBReq_enum_ovrdval
  VVMC_ADASAEBSta_enum_Inproc : FVT_lib/outp/OverrideAndLimit  SystemSampleTime=-1  VariantActivationTime=update diagram  Latency=0  AutoFrameSizeCalculation=off
      link override Signal_Limit/_maxval: Value=KOUTP_ADASAEBSta_enum_maxval
      link override Signal_Limit/_minval: Value=KOUTP_ADASAEBSta_enum_minval
      link override Signal_Override/_ovrdflg: Value=KOUTP_ADASAEBSta_enum_ovrdflg
      link override Signal_Override/_ovrdval: Value=KOUTP_ADASAEBSta_enum_ovrdval
  VVMC_ADASCAMSpdLim_enum_Inproc : FVT_lib/outp/OverrideAndLimit  SystemSampleTime=-1  VariantActivationTime=update diagram  Latency=0  AutoFrameSizeCalculation=off
      link override Signal_Limit/_maxval: Value=KOUTP_ADASCAMSpdLim_enum_maxval
      link override Signal_Limit/_minval: Value=KOUTP_ADASCAMSpdLim_enum_minval
      link override Signal_Override/_ovrdflg: Value=KOUTP_ADASCAMSpdLim_enum_ovrdflg
      link override Signal_Override/_ovrdval: Value=KOUTP_ADASCAMSpdLim_enum_ovrdval
  VVMC_ADASDBSReq_enum_Inproc : FVT_lib/outp/OverrideAndLimit  SystemSampleTime=-1  VariantActivationTime=update diagram  Latency=0  AutoFrameSizeCalculation=off
      link override Signal_Limit/_maxval: Value=KOUTP_ADASDBSReq_enum_maxval
      link override Signal_Limit/_minval: Value=KOUTP_ADASDBSReq_enum_minval
      link override Signal_Override/_ovrdflg: Value=KOUTP_ADASDBSReq_enum_ovrdflg
      link override Signal_Override/_ovrdval: Value=KOUTP_ADASDBSReq_enum_ovrdval
  VVMC_ADASFCWMute_flg_Inproc : FVT_lib/outp/OverrideAndLimit  SystemSampleTime=-1  VariantActivationTime=update diagram  Latency=0  AutoFrameSizeCalculation=off
      link override Signal_Limit/_maxval: Value=KOUTP_ADASFCWMute_flg_maxval
      link override Signal_Limit/_minval: Value=KOUTP_ADASFCWMute_flg_minval
      link override Signal_Override/_ovrdflg: Value=KOUTP_ADASFCWMute_flg_ovrdflg
      link override Signal_Override/_ovrdval: Value=KOUTP_ADASFCWMute_flg_ovrdval
  VVMC_ADASFCWSta_enum_Inproc : FVT_lib/outp/OverrideAndLimit  SystemSampleTime=-1  VariantActivationTime=update diagram  Latency=0  AutoFrameSizeCalculation=off
      link override Signal_Limit/_maxval: Value=KOUTP_ADASFCWSta_enum_maxval
      link override Signal_Limit/_minval: Value=KOUTP_ADASFCWSta_enum_minval
      link override Signal_Override/_ovrdflg: Value=KOUTP_ADASFCWSta_enum_ovrdflg
      link override Signal_Override/_ovrdval: Value=KOUTP_ADASFCWSta_enum_ovrdval
  VVMC_ADASFaultSta_flg_Inproc : FVT_lib/outp/OverrideAndLimit  SystemSampleTime=-1  VariantActivationTime=update diagram  Latency=0  AutoFrameSizeCalculation=off
      link override Signal_Limit/_maxval: Value=KOUTP_ADASFaultSta_flg_maxval
      link override Signal_Limit/_minval: Value=KOUTP_ADASFaultSta_flg_minval
      link override Signal_Override/_ovrdflg: Value=KOUTP_ADASFaultSta_flg_ovrdflg
      link override Signal_Override/_ovrdval: Value=KOUTP_ADASFaultSta_flg_ovrdval
  VVMC_ADASFltWrnReq_flg_Inproc : FVT_lib/outp/OverrideAndLimit  SystemSampleTime=-1  VariantActivationTime=update diagram  Latency=0  AutoFrameSizeCalculation=off
      link override Signal_Limit/_maxval: Value=KOUTP_ADASFltWrnReq_flg_maxval
      link override Signal_Limit/_minval: Value=KOUTP_ADASFltWrnReq_flg_minval
      link override Signal_Override/_ovrdflg: Value=KOUTP_ADASFltWrnReq_flg_ovrdflg
      link override Signal_Override/_ovrdval: Value=KOUTP_ADASFltWrnReq_flg_ovrdval
  VVMC_ADASForceIdle_flg_Inproc : FVT_lib/outp/OverrideAndLimit  SystemSampleTime=-1  VariantActivationTime=update diagram  Latency=0  AutoFrameSizeCalculation=off
      link override Signal_Limit/_maxval: Value=KOUTP_ADASForceIdle_flg_maxval
      link override Signal_Limit/_minval: Value=KOUTP_ADASForceIdle_flg_minval
      link override Signal_Override/_ovrdflg: Value=KOUTP_ADASForceIdle_flg_ovrdflg
      link override Signal_Override/_ovrdval: Value=KOUTP_ADASForceIdle_flg_ovrdval
  VVMC_ADASISASta_enum_Inproc : FVT_lib/outp/OverrideAndLimit  SystemSampleTime=-1  VariantActivationTime=update diagram  Latency=0  AutoFrameSizeCalculation=off
      link override Signal_Limit/_maxval: Value=KOUTP_ADASISASta_enum_maxval
      link override Signal_Limit/_minval: Value=KOUTP_ADASISASta_enum_minval
      link override Signal_Override/_ovrdflg: Value=KOUTP_ADASISASta_enum_ovrdflg
      link override Signal_Override/_ovrdval: Value=KOUTP_ADASISASta_enum_ovrdval
  VVMC_ADASLDWMute_flg_Inproc : FVT_lib/outp/OverrideAndLimit  SystemSampleTime=-1  VariantActivationTime=update diagram  Latency=0  AutoFrameSizeCalculation=off
      link override Signal_Limit/_maxval: Value=KOUTP_ADASLDWMute_flg_maxval
      link override Signal_Limit/_minval: Value=KOUTP_ADASLDWMute_flg_minval
      link override Signal_Override/_ovrdflg: Value=KOUTP_ADASLDWMute_flg_ovrdflg
      link override Signal_Override/_ovrdval: Value=KOUTP_ADASLDWMute_flg_ovrdval
  VVMC_ADASLDWSta_enum_Inproc : FVT_lib/outp/OverrideAndLimit  SystemSampleTime=-1  VariantActivationTime=update diagram  Latency=0  AutoFrameSizeCalculation=off
      link override Signal_Limit/_maxval: Value=KOUTP_ADASLDWSta_enum_maxval
      link override Signal_Limit/_minval: Value=KOUTP_ADASLDWSta_enum_minval
      link override Signal_Override/_ovrdflg: Value=KOUTP_ADASLDWSta_enum_ovrdflg
      link override Signal_Override/_ovrdval: Value=KOUTP_ADASLDWSta_enum_ovrdval
  VVMC_ADASLFCHandsOffWarning_enum_Inproc : FVT_lib/outp/OverrideAndLimit  SystemSampleTime=-1  VariantActivationTime=update diagram  Latency=0  AutoFrameSizeCalculation=off
      link override Signal_Limit/_maxval: Value=KOUTP_ADASLFCHandsOffWarning_enum_maxval
      link override Signal_Limit/_minval: Value=KOUTP_ADASLFCHandsOffWarning_enum_minval
      link override Signal_Override/_ovrdflg: Value=KOUTP_ADASLFCHandsOffWarning_enum_ovrdflg
      link override Signal_Override/_ovrdval: Value=KOUTP_ADASLFCHandsOffWarning_enum_ovrdval
  VVMC_ADASLFCSta_enum_Inproc : FVT_lib/outp/OverrideAndLimit  SystemSampleTime=-1  VariantActivationTime=update diagram  Latency=0  AutoFrameSizeCalculation=off
      link override Signal_Limit/_maxval: Value=KOUTP_ADASLFCSta_enum_maxval
      link override Signal_Limit/_minval: Value=KOUTP_ADASLFCSta_enum_minval
      link override Signal_Override/_ovrdflg: Value=KOUTP_ADASLFCSta_enum_ovrdflg
      link override Signal_Override/_ovrdval: Value=KOUTP_ADASLFCSta_enum_ovrdval
  VVMC_ADASLFCWarnSound_enum_Inproc : FVT_lib/outp/OverrideAndLimit  SystemSampleTime=-1  VariantActivationTime=update diagram  Latency=0  AutoFrameSizeCalculation=off
      link override Signal_Limit/_maxval: Value=KOUTP_ADASLFCWarnSound_enum_maxval
      link override Signal_Limit/_minval: Value=KOUTP_ADASLFCWarnSound_enum_minval
      link override Signal_Override/_ovrdflg: Value=KOUTP_ADASLFCWarnSound_enum_ovrdflg
      link override Signal_Override/_ovrdval: Value=KOUTP_ADASLFCWarnSound_enum_ovrdval
  VVMC_ADASLKASta_enum_Inproc : FVT_lib/outp/OverrideAndLimit  SystemSampleTime=-1  VariantActivationTime=update diagram  Latency=0  AutoFrameSizeCalculation=off
      link override Signal_Limit/_maxval: Value=KOUTP_ADASLKASta_enum_maxval
      link override Signal_Limit/_minval: Value=KOUTP_ADASLKASta_enum_minval
      link override Signal_Override/_ovrdflg: Value=KOUTP_ADASLKASta_enum_ovrdflg
      link override Signal_Override/_ovrdval: Value=KOUTP_ADASLKASta_enum_ovrdval
  VVMC_ADASLaneModeL_enum_Inproc : FVT_lib/outp/OverrideAndLimit  SystemSampleTime=-1  VariantActivationTime=update diagram  Latency=0  AutoFrameSizeCalculation=off
      link override Signal_Limit/_maxval: Value=KOUTP_ADASLaneModeL_enum_maxval
      link override Signal_Limit/_minval: Value=KOUTP_ADASLaneModeL_enum_minval
      link override Signal_Override/_ovrdflg: Value=KOUTP_ADASLaneModeL_enum_ovrdflg
      link override Signal_Override/_ovrdval: Value=KOUTP_ADASLaneModeL_enum_ovrdval
  VVMC_ADASLaneModeR_enum_Inproc : FVT_lib/outp/OverrideAndLimit  SystemSampleTime=-1  VariantActivationTime=update diagram  Latency=0  AutoFrameSizeCalculation=off
      link override Signal_Limit/_maxval: Value=KOUTP_ADASLaneModeR_enum_maxval
      link override Signal_Limit/_minval: Value=KOUTP_ADASLaneModeR_enum_minval
      link override Signal_Override/_ovrdflg: Value=KOUTP_ADASLaneModeR_enum_ovrdflg
      link override Signal_Override/_ovrdval: Value=KOUTP_ADASLaneModeR_enum_ovrdval
  VVMC_ADASLanecurveL_raw32_Inproc : FVT_lib/outp/OverrideAndLimit  SystemSampleTime=-1  VariantActivationTime=update diagram  Latency=0  AutoFrameSizeCalculation=off
      link override Signal_Limit/_maxval: Value=KOUTP_ADASLanecurveL_raw32_maxval
      link override Signal_Limit/_minval: Value=KOUTP_ADASLanecurveL_raw32_minval
      link override Signal_Override/_ovrdflg: Value=KOUTP_ADASLanecurveL_raw32_ovrdflg
      link override Signal_Override/_ovrdval: Value=KOUTP_ADASLanecurveL_raw32_ovrdval
  VVMC_ADASLanecurveR_raw32_Inproc : FVT_lib/outp/OverrideAndLimit  SystemSampleTime=-1  VariantActivationTime=update diagram  Latency=0  AutoFrameSizeCalculation=off
      link override Signal_Limit/_maxval: Value=KOUTP_ADASLanecurveR_raw32_maxval
      link override Signal_Limit/_minval: Value=KOUTP_ADASLanecurveR_raw32_minval
      link override Signal_Override/_ovrdflg: Value=KOUTP_ADASLanecurveR_raw32_ovrdflg
      link override Signal_Override/_ovrdval: Value=KOUTP_ADASLanecurveR_raw32_ovrdval
  VVMC_ADASLanetypeL_enum_Inproc : FVT_lib/outp/OverrideAndLimit  SystemSampleTime=-1  VariantActivationTime=update diagram  Latency=0  AutoFrameSizeCalculation=off
      link override Signal_Limit/_maxval: Value=KOUTP_ADASLanetypeL_enum_maxval
      link override Signal_Limit/_minval: Value=KOUTP_ADASLanetypeL_enum_minval
      link override Signal_Override/_ovrdflg: Value=KOUTP_ADASLanetypeL_enum_ovrdflg
      link override Signal_Override/_ovrdval: Value=KOUTP_ADASLanetypeL_enum_ovrdval
  VVMC_ADASLanetypeR_enum_Inproc : FVT_lib/outp/OverrideAndLimit  SystemSampleTime=-1  VariantActivationTime=update diagram  Latency=0  AutoFrameSizeCalculation=off
      link override Signal_Limit/_maxval: Value=KOUTP_ADASLanetypeR_enum_maxval
      link override Signal_Limit/_minval: Value=KOUTP_ADASLanetypeR_enum_minval
      link override Signal_Override/_ovrdflg: Value=KOUTP_ADASLanetypeR_enum_ovrdflg
      link override Signal_Override/_ovrdval: Value=KOUTP_ADASLanetypeR_enum_ovrdval
  VVMC_ADASSLIFSpdLim_enum_Inproc : FVT_lib/outp/OverrideAndLimit  SystemSampleTime=-1  VariantActivationTime=update diagram  Latency=0  AutoFrameSizeCalculation=off
      link override Signal_Limit/_maxval: Value=KOUTP_ADASSLIFSpdLim_enum_maxval
      link override Signal_Limit/_minval: Value=KOUTP_ADASSLIFSpdLim_enum_minval
      link override Signal_Override/_ovrdflg: Value=KOUTP_ADASSLIFSpdLim_enum_ovrdflg
      link override Signal_Override/_ovrdval: Value=KOUTP_ADASSLIFSpdLim_enum_ovrdval
  VVMC_ADASSLIFSta_enum_Inproc : FVT_lib/outp/OverrideAndLimit  SystemSampleTime=-1  VariantActivationTime=update diagram  Latency=0  AutoFrameSizeCalculation=off
      link override Signal_Limit/_maxval: Value=KOUTP_ADASSLIFSta_enum_maxval
      link override Signal_Limit/_minval: Value=KOUTP_ADASSLIFSta_enum_minval
      link override Signal_Override/_ovrdflg: Value=KOUTP_ADASSLIFSta_enum_ovrdflg
      link override Signal_Override/_ovrdval: Value=KOUTP_ADASSLIFSta_enum_ovrdval
  VVMC_ADASShftPosnReqA_flg_Inproc : FVT_lib/outp/OverrideAndLimit  SystemSampleTime=-1  VariantActivationTime=update diagram  Latency=0  AutoFrameSizeCalculation=off
      link override Signal_Limit/_maxval: Value=KOUTP_ADASShftPosnReqA_flg_maxval
      link override Signal_Limit/_minval: Value=KOUTP_ADASShftPosnReqA_flg_minval
      link override Signal_Override/_ovrdflg: Value=KOUTP_ADASShftPosnReqA_flg_ovrdflg
      link override Signal_Override/_ovrdval: Value=KOUTP_ADASShftPosnReqA_flg_ovrdval
  VVMC_ADASShftPosnReq_enum_Inproc : FVT_lib/outp/OverrideAndLimit  SystemSampleTime=-1  VariantActivationTime=update diagram  Latency=0  AutoFrameSizeCalculation=off
      link override Signal_Limit/_maxval: Value=KOUTP_ADASShftPosnReq_enum_maxval
      link override Signal_Limit/_minval: Value=KOUTP_ADASShftPosnReq_enum_minval
      link override Signal_Override/_ovrdflg: Value=KOUTP_ADASShftPosnReq_enum_ovrdflg
      link override Signal_Override/_ovrdval: Value=KOUTP_ADASShftPosnReq_enum_ovrdval
  VVMC_ADASVehSpdLim_raw32_Inproc : FVT_lib/outp/OverrideAndLimit  SystemSampleTime=-1  VariantActivationTime=update diagram  Latency=0  AutoFrameSizeCalculation=off
      link override Signal_Limit/_maxval: Value=KOUTP_ADASVehSpdLim_raw32_maxval
      link override Signal_Limit/_minval: Value=KOUTP_ADASVehSpdLim_raw32_minval
      link override Signal_Override/_ovrdflg: Value=KOUTP_ADASVehSpdLim_raw32_ovrdflg
      link override Signal_Override/_ovrdval: Value=KOUTP_ADASVehSpdLim_raw32_ovrdval
  VVMC_ADASWarningMsg_enum_Inproc : FVT_lib/outp/OverrideAndLimit  SystemSampleTime=-1  VariantActivationTime=update diagram  Latency=0  AutoFrameSizeCalculation=off
      link override Signal_Limit/_maxval: Value=KOUTP_ADASWarningMsg_enum_maxval
      link override Signal_Limit/_minval: Value=KOUTP_ADASWarningMsg_enum_minval
      link override Signal_Override/_ovrdflg: Value=KOUTP_ADASWarningMsg_enum_ovrdflg
      link override Signal_Override/_ovrdval: Value=KOUTP_ADASWarningMsg_enum_ovrdval
  VVMC_AEBVehHoldReq_flg_Inproc : FVT_lib/outp/OverrideAndLimit  SystemSampleTime=-1  VariantActivationTime=update diagram  Latency=0  AutoFrameSizeCalculation=off
      link override Signal_Limit/_maxval: Value=KOUTP_AEBVehHoldReq_flg_maxval
      link override Signal_Limit/_minval: Value=KOUTP_AEBVehHoldReq_flg_minval
      link override Signal_Override/_ovrdflg: Value=KOUTP_AEBVehHoldReq_flg_ovrdflg
      link override Signal_Override/_ovrdval: Value=KOUTP_AEBVehHoldReq_flg_ovrdval
  VVMC_APSActive_flg_Inproc : FVT_lib/outp/OverrideAndLimit  SystemSampleTime=-1  VariantActivationTime=update diagram  Latency=0  AutoFrameSizeCalculation=off
      link override Signal_Limit/_maxval: Value=KOUTP_APSActive_flg_maxval
      link override Signal_Limit/_minval: Value=KOUTP_APSActive_flg_minval
      link override Signal_Override/_ovrdflg: Value=KOUTP_APSActive_flg_ovrdflg
      link override Signal_Override/_ovrdval: Value=KOUTP_APSActive_flg_ovrdval
  VVMC_APSCtrlAvail_flg_Inproc : FVT_lib/outp/OverrideAndLimit  SystemSampleTime=-1  VariantActivationTime=update diagram  Latency=0  AutoFrameSizeCalculation=off
      link override Signal_Limit/_maxval: Value=KOUTP_APSCtrlAvail_flg_maxval
      link override Signal_Limit/_minval: Value=KOUTP_APSCtrlAvail_flg_minval
      link override Signal_Override/_ovrdflg: Value=KOUTP_APSCtrlAvail_flg_ovrdflg
      link override Signal_Override/_ovrdval: Value=KOUTP_APSCtrlAvail_flg_ovrdval
  VVMC_APSDecReqA_flg_Inproc : FVT_lib/outp/OverrideAndLimit  SystemSampleTime=-1  VariantActivationTime=update diagram  Latency=0  AutoFrameSizeCalculation=off
      link override Signal_Limit/_maxval: Value=KOUTP_APSDecReqA_flg_maxval
      link override Signal_Limit/_minval: Value=KOUTP_APSDecReqA_flg_minval
      link override Signal_Override/_ovrdflg: Value=KOUTP_APSDecReqA_flg_ovrdflg
      link override Signal_Override/_ovrdval: Value=KOUTP_APSDecReqA_flg_ovrdval
  VVMC_APSDecReq_mps2_Inproc : FVT_lib/outp/OverrideAndLimit  SystemSampleTime=-1  VariantActivationTime=update diagram  Latency=0  AutoFrameSizeCalculation=off
      link override Signal_Limit/_maxval: Value=KOUTP_APSDecReq_mps2_maxval
      link override Signal_Limit/_minval: Value=KOUTP_APSDecReq_mps2_minval
      link override Signal_Override/_ovrdflg: Value=KOUTP_APSDecReq_mps2_ovrdflg
      link override Signal_Override/_ovrdval: Value=KOUTP_APSDecReq_mps2_ovrdval
  VVMC_APSReq_enum_Inproc : FVT_lib/outp/OverrideAndLimit  SystemSampleTime=-1  VariantActivationTime=update diagram  Latency=0  AutoFrameSizeCalculation=off
      link override Signal_Limit/_maxval: Value=KOUTP_APSReq_enum_maxval
      link override Signal_Limit/_minval: Value=KOUTP_APSReq_enum_minval
      link override Signal_Override/_ovrdflg: Value=KOUTP_APSReq_enum_ovrdflg
      link override Signal_Override/_ovrdval: Value=KOUTP_APSReq_enum_ovrdval
  VVMC_APSStaSys_enum_Inproc : FVT_lib/outp/OverrideAndLimit  SystemSampleTime=-1  VariantActivationTime=update diagram  Latency=0  AutoFrameSizeCalculation=off
      link override Signal_Limit/_maxval: Value=KOUTP_APSStaSys_enum_maxval
      link override Signal_Limit/_minval: Value=KOUTP_APSStaSys_enum_minval
      link override Signal_Override/_ovrdflg: Value=KOUTP_APSStaSys_enum_ovrdflg
      link override Signal_Override/_ovrdval: Value=KOUTP_APSStaSys_enum_ovrdval
  VVMC_AccCalcuPID_mps2_Inproc : FVT_lib/outp/OverrideAndLimit  SystemSampleTime=-1  VariantActivationTime=update diagram  Latency=0  AutoFrameSizeCalculation=off
      link override Signal_Limit/_maxval: Value=KOUTP_AccCalcuPID_mps2_maxval
      link override Signal_Limit/_minval: Value=KOUTP_AccCalcuPID_mps2_minval
      link override Signal_Override/_ovrdflg: Value=KOUTP_AccCalcuPID_mps2_ovrdflg
      link override Signal_Override/_ovrdval: Value=KOUTP_AccCalcuPID_mps2_ovrdval
  VVMC_ActACCRequiredAccel_mps2_Inproc : FVT_lib/outp/OverrideAndLimit  SystemSampleTime=-1  VariantActivationTime=update diagram  Latency=0  AutoFrameSizeCalculation=off
      link override Signal_Limit/_maxval: Value=KOUTP_ActACCRequiredAccel_mps2_maxval
      link override Signal_Limit/_minval: Value=KOUTP_ActACCRequiredAccel_mps2_minval
      link override Signal_Override/_ovrdflg: Value=KOUTP_ActACCRequiredAccel_mps2_ovrdflg
      link override Signal_Override/_ovrdval: Value=KOUTP_ActACCRequiredAccel_mps2_ovrdval
  VVMC_CAASActive_flg_Inproc : FVT_lib/outp/OverrideAndLimit  SystemSampleTime=-1  VariantActivationTime=update diagram  Latency=0  AutoFrameSizeCalculation=off
      link override Signal_Limit/_maxval: Value=KOUTP_CAASActive_flg_maxval
      link override Signal_Limit/_minval: Value=KOUTP_CAASActive_flg_minval
      link override Signal_Override/_ovrdflg: Value=KOUTP_CAASActive_flg_ovrdflg
      link override Signal_Override/_ovrdval: Value=KOUTP_CAASActive_flg_ovrdval
  VVMC_CAASCtrlAvail_flg_Inproc : FVT_lib/outp/OverrideAndLimit  SystemSampleTime=-1  VariantActivationTime=update diagram  Latency=0  AutoFrameSizeCalculation=off
      link override Signal_Limit/_maxval: Value=KOUTP_CAASCtrlAvail_flg_maxval
      link override Signal_Limit/_minval: Value=KOUTP_CAASCtrlAvail_flg_minval
      link override Signal_Override/_ovrdflg: Value=KOUTP_CAASCtrlAvail_flg_ovrdflg
      link override Signal_Override/_ovrdval: Value=KOUTP_CAASCtrlAvail_flg_ovrdval
  VVMC_CCCtrlSta_enum_Inproc : FVT_lib/outp/OverrideAndLimit  SystemSampleTime=-1  VariantActivationTime=update diagram  Latency=0  AutoFrameSizeCalculation=off
      link override Signal_Limit/_maxval: Value=KOUTP_CCCtrlSta_enum_maxval
      link override Signal_Limit/_minval: Value=KOUTP_CCCtrlSta_enum_minval
      link override Signal_Override/_ovrdflg: Value=KOUTP_CCCtrlSta_enum_ovrdflg
      link override Signal_Override/_ovrdval: Value=KOUTP_CCCtrlSta_enum_ovrdval
  VVMC_CCMSASpdWar_flg_Inproc : FVT_lib/outp/OverrideAndLimit  SystemSampleTime=-1  VariantActivationTime=update diagram  Latency=0  AutoFrameSizeCalculation=off
      link override Signal_Limit/_maxval: Value=KOUTP_CCMSASpdWar_flg_maxval
      link override Signal_Limit/_minval: Value=KOUTP_CCMSASpdWar_flg_minval
      link override Signal_Override/_ovrdflg: Value=KOUTP_CCMSASpdWar_flg_ovrdflg
      link override Signal_Override/_ovrdval: Value=KOUTP_CCMSASpdWar_flg_ovrdval
  VVMC_CalibratedAccX_G_Inproc : FVT_lib/outp/OverrideAndLimit  SystemSampleTime=-1  VariantActivationTime=update diagram  Latency=0  AutoFrameSizeCalculation=off
      link override Signal_Limit/_maxval: Value=KOUTP_CalibratedAccX_G_maxval
      link override Signal_Limit/_minval: Value=KOUTP_CalibratedAccX_G_minval
      link override Signal_Override/_ovrdflg: Value=KOUTP_CalibratedAccX_G_ovrdflg
      link override Signal_Override/_ovrdval: Value=KOUTP_CalibratedAccX_G_ovrdval
  VVMC_CalibratedAccY_G_Inproc : FVT_lib/outp/OverrideAndLimit  SystemSampleTime=-1  VariantActivationTime=update diagram  Latency=0  AutoFrameSizeCalculation=off
      link override Signal_Limit/_maxval: Value=KOUTP_CalibratedAccY_G_maxval
      link override Signal_Limit/_minval: Value=KOUTP_CalibratedAccY_G_minval
      link override Signal_Override/_ovrdflg: Value=KOUTP_CalibratedAccY_G_ovrdflg
      link override Signal_Override/_ovrdval: Value=KOUTP_CalibratedAccY_G_ovrdval
  VVMC_CalibratedAccZ_G_Inproc : FVT_lib/outp/OverrideAndLimit  SystemSampleTime=-1  VariantActivationTime=update diagram  Latency=0  AutoFrameSizeCalculation=off
      link override Signal_Limit/_maxval: Value=KOUTP_CalibratedAccZ_G_maxval
      link override Signal_Limit/_minval: Value=KOUTP_CalibratedAccZ_G_minval
      link override Signal_Override/_ovrdflg: Value=KOUTP_CalibratedAccZ_G_ovrdflg
      link override Signal_Override/_ovrdval: Value=KOUTP_CalibratedAccZ_G_ovrdval
  VVMC_CalibratedGyroX_Dps_Inproc : FVT_lib/outp/OverrideAndLimit  SystemSampleTime=-1  VariantActivationTime=update diagram  Latency=0  AutoFrameSizeCalculation=off
      link override Signal_Limit/_maxval: Value=KOUTP_CalibratedGyroX_Dps_maxval
      link override Signal_Limit/_minval: Value=KOUTP_CalibratedGyroX_Dps_minval
      link override Signal_Override/_ovrdflg: Value=KOUTP_CalibratedGyroX_Dps_ovrdflg
      link override Signal_Override/_ovrdval: Value=KOUTP_CalibratedGyroX_Dps_ovrdval
  VVMC_CalibratedGyroY_Dps_Inproc : FVT_lib/outp/OverrideAndLimit  SystemSampleTime=-1  VariantActivationTime=update diagram  Latency=0  AutoFrameSizeCalculation=off
      link override Signal_Limit/_maxval: Value=KOUTP_CalibratedGyroY_Dps_maxval
      link override Signal_Limit/_minval: Value=KOUTP_CalibratedGyroY_Dps_minval
      link override Signal_Override/_ovrdflg: Value=KOUTP_CalibratedGyroY_Dps_ovrdflg
      link override Signal_Override/_ovrdval: Value=KOUTP_CalibratedGyroY_Dps_ovrdval
  VVMC_CalibratedGyroZ_Dps_Inproc : FVT_lib/outp/OverrideAndLimit  SystemSampleTime=-1  VariantActivationTime=update diagram  Latency=0  AutoFrameSizeCalculation=off
      link override Signal_Limit/_maxval: Value=KOUTP_CalibratedGyroZ_Dps_maxval
      link override Signal_Limit/_minval: Value=KOUTP_CalibratedGyroZ_Dps_minval
      link override Signal_Override/_ovrdflg: Value=KOUTP_CalibratedGyroZ_Dps_ovrdflg
      link override Signal_Override/_ovrdval: Value=KOUTP_CalibratedGyroZ_Dps_ovrdval
  VVMC_DISCReqAcc_mps2_Inproc : FVT_lib/outp/OverrideAndLimit  SystemSampleTime=-1  VariantActivationTime=update diagram  Latency=0  AutoFrameSizeCalculation=off
      link override Signal_Limit/_maxval: Value=KOUTP_DISCReqAcc_mps2_maxval
      link override Signal_Limit/_minval: Value=KOUTP_DISCReqAcc_mps2_minval
      link override Signal_Override/_ovrdflg: Value=KOUTP_DISCReqAcc_mps2_ovrdflg
      link override Signal_Override/_ovrdval: Value=KOUTP_DISCReqAcc_mps2_ovrdval
  VVMC_ExtraMSACtrlSta_enum_Inproc : FVT_lib/outp/OverrideAndLimit  SystemSampleTime=-1  VariantActivationTime=update diagram  Latency=0  AutoFrameSizeCalculation=off
      link override Signal_Limit/_maxval: Value=KOUTP_ExtraMSACtrlSta_enum_maxval
      link override Signal_Limit/_minval: Value=KOUTP_ExtraMSACtrlSta_enum_minval
      link override Signal_Override/_ovrdflg: Value=KOUTP_ExtraMSACtrlSta_enum_ovrdflg
      link override Signal_Override/_ovrdval: Value=KOUTP_ExtraMSACtrlSta_enum_ovrdval
  VVMC_FCMACCmode_enum_Inproc : FVT_lib/outp/OverrideAndLimit  SystemSampleTime=-1  VariantActivationTime=update diagram  Latency=0  AutoFrameSizeCalculation=off
      link override Signal_Limit/_maxval: Value=KOUTP_FCMACCmode_enum_maxval
      link override Signal_Limit/_minval: Value=KOUTP_FCMACCmode_enum_minval
      link override Signal_Override/_ovrdflg: Value=KOUTP_FCMACCmode_enum_ovrdflg
      link override Signal_Override/_ovrdval: Value=KOUTP_FCMACCmode_enum_ovrdval
  VVMC_FCMLDWFault_flg_Inproc : FVT_lib/outp/OverrideAndLimit  SystemSampleTime=-1  VariantActivationTime=update diagram  Latency=0  AutoFrameSizeCalculation=off
      link override Signal_Limit/_maxval: Value=KOUTP_FCMLDWFault_flg_maxval
      link override Signal_Limit/_minval: Value=KOUTP_FCMLDWFault_flg_minval
      link override Signal_Override/_ovrdflg: Value=KOUTP_FCMLDWFault_flg_ovrdflg
      link override Signal_Override/_ovrdval: Value=KOUTP_FCMLDWFault_flg_ovrdval
  VVMC_FCMLDWRequest_enum_Inproc : FVT_lib/outp/OverrideAndLimit  SystemSampleTime=-1  VariantActivationTime=update diagram  Latency=0  AutoFrameSizeCalculation=off
      link override Signal_Limit/_maxval: Value=KOUTP_FCMLDWRequest_enum_maxval
      link override Signal_Limit/_minval: Value=KOUTP_FCMLDWRequest_enum_minval
      link override Signal_Override/_ovrdflg: Value=KOUTP_FCMLDWRequest_enum_ovrdflg
      link override Signal_Override/_ovrdval: Value=KOUTP_FCMLDWRequest_enum_ovrdval
  VVMC_FDCVMCAPSAngleTarget_deg_Inproc : FVT_lib/outp/OverrideAndLimit  SystemSampleTime=-1  VariantActivationTime=update diagram  Latency=0  AutoFrameSizeCalculation=off
      link override Signal_Limit/_maxval: Value=KOUTP_FDCVMCAPSAngleTarget_deg_maxval
      link override Signal_Limit/_minval: Value=KOUTP_FDCVMCAPSAngleTarget_deg_minval
      link override Signal_Override/_ovrdflg: Value=KOUTP_FDCVMCAPSAngleTarget_deg_ovrdflg
      link override Signal_Override/_ovrdval: Value=KOUTP_FDCVMCAPSAngleTarget_deg_ovrdval
  VVMC_FDCVMCAPSRqEPSCtrl_flg_Inproc : FVT_lib/outp/OverrideAndLimit  SystemSampleTime=-1  VariantActivationTime=update diagram  Latency=0  AutoFrameSizeCalculation=off
      link override Signal_Limit/_maxval: Value=KOUTP_FDCVMCAPSRqEPSCtrl_flg_maxval
      link override Signal_Limit/_minval: Value=KOUTP_FDCVMCAPSRqEPSCtrl_flg_minval
      link override Signal_Override/_ovrdflg: Value=KOUTP_FDCVMCAPSRqEPSCtrl_flg_ovrdflg
      link override Signal_Override/_ovrdval: Value=KOUTP_FDCVMCAPSRqEPSCtrl_flg_ovrdval
  VVMC_FDCVMCAPSVRqEPSCtrl_flg_Inproc : FVT_lib/outp/OverrideAndLimit  SystemSampleTime=-1  VariantActivationTime=update diagram  Latency=0  AutoFrameSizeCalculation=off
      link override Signal_Limit/_maxval: Value=KOUTP_FDCVMCAPSVRqEPSCtrl_flg_maxval
      link override Signal_Limit/_minval: Value=KOUTP_FDCVMCAPSVRqEPSCtrl_flg_minval
      link override Signal_Override/_ovrdflg: Value=KOUTP_FDCVMCAPSVRqEPSCtrl_flg_ovrdflg
      link override Signal_Override/_ovrdval: Value=KOUTP_FDCVMCAPSVRqEPSCtrl_flg_ovrdval
  VVMC_FDCVMCAngCtrlTqWtGn_pct_Inproc : FVT_lib/outp/OverrideAndLimit  SystemSampleTime=-1  VariantActivationTime=update diagram  Latency=0  AutoFrameSizeCalculation=off
      link override Signal_Limit/_maxval: Value=KOUTP_FDCVMCAngCtrlTqWtGn_pct_maxval
      link override Signal_Limit/_minval: Value=KOUTP_FDCVMCAngCtrlTqWtGn_pct_minval
      link override Signal_Override/_ovrdflg: Value=KOUTP_FDCVMCAngCtrlTqWtGn_pct_ovrdflg
      link override Signal_Override/_ovrdval: Value=KOUTP_FDCVMCAngCtrlTqWtGn_pct_ovrdval
  VVMC_FDCVMCDrInpTqBstAct_flg_Inproc : FVT_lib/outp/OverrideAndLimit  SystemSampleTime=-1  VariantActivationTime=update diagram  Latency=0  AutoFrameSizeCalculation=off
      link override Signal_Limit/_maxval: Value=KOUTP_FDCVMCDrInpTqBstAct_flg_maxval
      link override Signal_Limit/_minval: Value=KOUTP_FDCVMCDrInpTqBstAct_flg_minval
      link override Signal_Override/_ovrdflg: Value=KOUTP_FDCVMCDrInpTqBstAct_flg_ovrdflg
      link override Signal_Override/_ovrdval: Value=KOUTP_FDCVMCDrInpTqBstAct_flg_ovrdval
  VVMC_FDCVMCDrInpTqBstGn_pct_Inproc : FVT_lib/outp/OverrideAndLimit  SystemSampleTime=-1  VariantActivationTime=update diagram  Latency=0  AutoFrameSizeCalculation=off
      link override Signal_Limit/_maxval: Value=KOUTP_FDCVMCDrInpTqBstGn_pct_maxval
      link override Signal_Limit/_minval: Value=KOUTP_FDCVMCDrInpTqBstGn_pct_minval
      link override Signal_Override/_ovrdflg: Value=KOUTP_FDCVMCDrInpTqBstGn_pct_ovrdflg
      link override Signal_Override/_ovrdval: Value=KOUTP_FDCVMCDrInpTqBstGn_pct_ovrdval
  VVMC_FDCVMCMaxAngCtrlOutTqLim_Nm_Inproc : FVT_lib/outp/OverrideAndLimit  SystemSampleTime=-1  VariantActivationTime=update diagram  Latency=0  AutoFrameSizeCalculation=off
      link override Signal_Limit/_maxval: Value=KOUTP_FDCVMCMaxAngCtrlOutTqLim_Nm_maxval
      link override Signal_Limit/_minval: Value=KOUTP_FDCVMCMaxAngCtrlOutTqLim_Nm_minval
      link override Signal_Override/_ovrdflg: Value=KOUTP_FDCVMCMaxAngCtrlOutTqLim_Nm_ovrdflg
      link override Signal_Override/_ovrdval: Value=KOUTP_FDCVMCMaxAngCtrlOutTqLim_Nm_ovrdval
  VVMC_FeatArbitrFinal_enum_Inproc : FVT_lib/outp/OverrideAndLimit  SystemSampleTime=-1  VariantActivationTime=update diagram  Latency=0  AutoFrameSizeCalculation=off
      link override Signal_Limit/_maxval: Value=KOUTP_FeatArbitrFinal_enum_maxval
      link override Signal_Limit/_minval: Value=KOUTP_FeatArbitrFinal_enum_minval
      link override Signal_Override/_ovrdflg: Value=KOUTP_FeatArbitrFinal_enum_ovrdflg
      link override Signal_Override/_ovrdval: Value=KOUTP_FeatArbitrFinal_enum_ovrdval
  VVMC_FeatArbitrSta_enum_Inproc : FVT_lib/outp/OverrideAndLimit  SystemSampleTime=-1  VariantActivationTime=update diagram  Latency=0  AutoFrameSizeCalculation=off
      link override Signal_Limit/_maxval: Value=KOUTP_FeatArbitrSta_enum_maxval
      link override Signal_Limit/_minval: Value=KOUTP_FeatArbitrSta_enum_minval
      link override Signal_Override/_ovrdflg: Value=KOUTP_FeatArbitrSta_enum_ovrdflg
      link override Signal_Override/_ovrdval: Value=KOUTP_FeatArbitrSta_enum_ovrdval
  VVMC_FeatReqSpd_kph_Inproc : FVT_lib/outp/OverrideAndLimit  SystemSampleTime=-1  VariantActivationTime=update diagram  Latency=0  AutoFrameSizeCalculation=off
      link override Signal_Limit/_maxval: Value=KOUTP_FeatReqSpd_kph_maxval
      link override Signal_Limit/_minval: Value=KOUTP_FeatReqSpd_kph_minval
      link override Signal_Override/_ovrdflg: Value=KOUTP_FeatReqSpd_kph_ovrdflg
      link override Signal_Override/_ovrdval: Value=KOUTP_FeatReqSpd_kph_ovrdval
  VVMC_FeatSetSpdFinal_raw32_Inproc : FVT_lib/outp/OverrideAndLimit  SystemSampleTime=-1  VariantActivationTime=update diagram  Latency=0  AutoFrameSizeCalculation=off
      link override Signal_Limit/_maxval: Value=KOUTP_FeatSetSpdFinal_raw32_maxval
      link override Signal_Limit/_minval: Value=KOUTP_FeatSetSpdFinal_raw32_minval
      link override Signal_Override/_ovrdflg: Value=KOUTP_FeatSetSpdFinal_raw32_ovrdflg
      link override Signal_Override/_ovrdval: Value=KOUTP_FeatSetSpdFinal_raw32_ovrdval
  VVMC_ForceLowBeam_enum_Inproc : FVT_lib/outp/OverrideAndLimit  SystemSampleTime=-1  VariantActivationTime=update diagram  Latency=0  AutoFrameSizeCalculation=off
      link override Signal_Limit/_maxval: Value=KOUTP_ForceLowBeam_enum_maxval
      link override Signal_Limit/_minval: Value=KOUTP_ForceLowBeam_enum_minval
      link override Signal_Override/_ovrdflg: Value=KOUTP_ForceLowBeam_enum_ovrdflg
      link override Signal_Override/_ovrdval: Value=KOUTP_ForceLowBeam_enum_ovrdval
  VVMC_FrontRearSlipRatioCtrl_flg_Inproc : FVT_lib/outp/OverrideAndLimit  SystemSampleTime=-1  VariantActivationTime=update diagram  Latency=0  AutoFrameSizeCalculation=off
      link override Signal_Limit/_maxval: Value=KOUTP_FrontRearSlipRatioCtrl_flg_maxval
      link override Signal_Limit/_minval: Value=KOUTP_FrontRearSlipRatioCtrl_flg_minval
      link override Signal_Override/_ovrdflg: Value=KOUTP_FrontRearSlipRatioCtrl_flg_ovrdflg
      link override Signal_Override/_ovrdval: Value=KOUTP_FrontRearSlipRatioCtrl_flg_ovrdval
  VVMC_HazardWarningReq_flg_Inproc : FVT_lib/outp/OverrideAndLimit  SystemSampleTime=-1  VariantActivationTime=update diagram  Latency=0  AutoFrameSizeCalculation=off
      link override Signal_Limit/_maxval: Value=KOUTP_HazardWarningReq_flg_maxval
      link override Signal_Limit/_minval: Value=KOUTP_HazardWarningReq_flg_minval
      link override Signal_Override/_ovrdflg: Value=KOUTP_HazardWarningReq_flg_ovrdflg
      link override Signal_Override/_ovrdval: Value=KOUTP_HazardWarningReq_flg_ovrdval
  VVMC_IMUEnaCmd_flg_Inproc : FVT_lib/outp/OverrideAndLimit  SystemSampleTime=-1  VariantActivationTime=update diagram  Latency=0  AutoFrameSizeCalculation=off
      link override Signal_Limit/_maxval: Value=KOUTP_IMUEnaCmd_flg_maxval
      link override Signal_Limit/_minval: Value=KOUTP_IMUEnaCmd_flg_minval
      link override Signal_Override/_ovrdflg: Value=KOUTP_IMUEnaCmd_flg_ovrdflg
      link override Signal_Override/_ovrdval: Value=KOUTP_IMUEnaCmd_flg_ovrdval
  VVMC_ISOAccLimit_mps2_Inproc : FVT_lib/outp/OverrideAndLimit  SystemSampleTime=-1  VariantActivationTime=update diagram  Latency=0  AutoFrameSizeCalculation=off
      link override Signal_Limit/_maxval: Value=KOUTP_ISOAccLimit_mps2_maxval
      link override Signal_Limit/_minval: Value=KOUTP_ISOAccLimit_mps2_minval
      link override Signal_Override/_ovrdflg: Value=KOUTP_ISOAccLimit_mps2_ovrdflg
      link override Signal_Override/_ovrdval: Value=KOUTP_ISOAccLimit_mps2_ovrdval
  VVMC_ISODecLimit_mps2_Inproc : FVT_lib/outp/OverrideAndLimit  SystemSampleTime=-1  VariantActivationTime=update diagram  Latency=0  AutoFrameSizeCalculation=off
      link override Signal_Limit/_maxval: Value=KOUTP_ISODecLimit_mps2_maxval
      link override Signal_Limit/_minval: Value=KOUTP_ISODecLimit_mps2_minval
      link override Signal_Override/_ovrdflg: Value=KOUTP_ISODecLimit_mps2_ovrdflg
      link override Signal_Override/_ovrdval: Value=KOUTP_ISODecLimit_mps2_ovrdval
  VVMC_ISOJerkLimit_mps3_Inproc : FVT_lib/outp/OverrideAndLimit  SystemSampleTime=-1  VariantActivationTime=update diagram  Latency=0  AutoFrameSizeCalculation=off
      link override Signal_Limit/_maxval: Value=KOUTP_ISOJerkLimit_mps3_maxval
      link override Signal_Limit/_minval: Value=KOUTP_ISOJerkLimit_mps3_minval
      link override Signal_Override/_ovrdflg: Value=KOUTP_ISOJerkLimit_mps3_ovrdflg
      link override Signal_Override/_ovrdval: Value=KOUTP_ISOJerkLimit_mps3_ovrdval
  VVMC_JerkPCT_pct_Inproc : FVT_lib/outp/OverrideAndLimit  SystemSampleTime=-1  VariantActivationTime=update diagram  Latency=0  AutoFrameSizeCalculation=off
      link override Signal_Limit/_maxval: Value=KOUTP_JerkPCT_pct_maxval
      link override Signal_Limit/_minval: Value=KOUTP_JerkPCT_pct_minval
      link override Signal_Override/_ovrdflg: Value=KOUTP_JerkPCT_pct_ovrdflg
      link override Signal_Override/_ovrdval: Value=KOUTP_JerkPCT_pct_ovrdval
  VVMC_LKAHODDisplayWarning_flg_Inproc : FVT_lib/outp/OverrideAndLimit  SystemSampleTime=-1  VariantActivationTime=update diagram  Latency=0  AutoFrameSizeCalculation=off
      link override Signal_Limit/_maxval: Value=KOUTP_LKAHODDisplayWarning_flg_maxval
      link override Signal_Limit/_minval: Value=KOUTP_LKAHODDisplayWarning_flg_minval
      link override Signal_Override/_ovrdflg: Value=KOUTP_LKAHODDisplayWarning_flg_ovrdflg
      link override Signal_Override/_ovrdval: Value=KOUTP_LKAHODDisplayWarning_flg_ovrdval
  VVMC_LKAHODSoundWarning_flg_Inproc : FVT_lib/outp/OverrideAndLimit  SystemSampleTime=-1  VariantActivationTime=update diagram  Latency=0  AutoFrameSizeCalculation=off
      link override Signal_Limit/_maxval: Value=KOUTP_LKAHODSoundWarning_flg_maxval
      link override Signal_Limit/_minval: Value=KOUTP_LKAHODSoundWarning_flg_minval
      link override Signal_Override/_ovrdflg: Value=KOUTP_LKAHODSoundWarning_flg_ovrdflg
      link override Signal_Override/_ovrdval: Value=KOUTP_LKAHODSoundWarning_flg_ovrdval
  VVMC_LKAStrToqReq_Nm_Inproc : FVT_lib/outp/OverrideAndLimit  SystemSampleTime=-1  VariantActivationTime=update diagram  Latency=0  AutoFrameSizeCalculation=off
      link override Signal_Limit/_maxval: Value=KOUTP_LKAStrToqReq_Nm_maxval
      link override Signal_Limit/_minval: Value=KOUTP_LKAStrToqReq_Nm_minval
      link override Signal_Override/_ovrdflg: Value=KOUTP_LKAStrToqReq_Nm_ovrdflg
      link override Signal_Override/_ovrdval: Value=KOUTP_LKAStrToqReq_Nm_ovrdval
  VVMC_LKATOIAct_enum_Inproc : FVT_lib/outp/OverrideAndLimit  SystemSampleTime=-1  VariantActivationTime=update diagram  Latency=0  AutoFrameSizeCalculation=off
      link override Signal_Limit/_maxval: Value=KOUTP_LKATOIAct_enum_maxval
      link override Signal_Limit/_minval: Value=KOUTP_LKATOIAct_enum_minval
      link override Signal_Override/_ovrdflg: Value=KOUTP_LKATOIAct_enum_ovrdflg
      link override Signal_Override/_ovrdval: Value=KOUTP_LKATOIAct_enum_ovrdval
  VVMC_LKATOIFault_flg_Inproc : FVT_lib/outp/OverrideAndLimit  SystemSampleTime=-1  VariantActivationTime=update diagram  Latency=0  AutoFrameSizeCalculation=off
      link override Signal_Limit/_maxval: Value=KOUTP_LKATOIFault_flg_maxval
      link override Signal_Limit/_minval: Value=KOUTP_LKATOIFault_flg_minval
      link override Signal_Override/_ovrdflg: Value=KOUTP_LKATOIFault_flg_ovrdflg
      link override Signal_Override/_ovrdval: Value=KOUTP_LKATOIFault_flg_ovrdval
  VVMC_LVDAACCStatusInformation_flg_Inproc : FVT_lib/outp/OverrideAndLimit  SystemSampleTime=-1  VariantActivationTime=update diagram  Latency=0  AutoFrameSizeCalculation=off
      link override Signal_Limit/_maxval: Value=KOUTP_LVDAACCStatusInformation_flg_maxval
      link override Signal_Limit/_minval: Value=KOUTP_LVDAACCStatusInformation_flg_minval
      link override Signal_Override/_ovrdflg: Value=KOUTP_LVDAACCStatusInformation_flg_ovrdflg
      link override Signal_Override/_ovrdval: Value=KOUTP_LVDAACCStatusInformation_flg_ovrdval
  VVMC_LVDADisabled_flg_Inproc : FVT_lib/outp/OverrideAndLimit  SystemSampleTime=-1  VariantActivationTime=update diagram  Latency=0  AutoFrameSizeCalculation=off
      link override Signal_Limit/_maxval: Value=KOUTP_LVDADisabled_flg_maxval
      link override Signal_Limit/_minval: Value=KOUTP_LVDADisabled_flg_minval
      link override Signal_Override/_ovrdflg: Value=KOUTP_LVDADisabled_flg_ovrdflg
      link override Signal_Override/_ovrdval: Value=KOUTP_LVDADisabled_flg_ovrdval
  VVMC_LVDAFailinfo_flg_Inproc : FVT_lib/outp/OverrideAndLimit  SystemSampleTime=-1  VariantActivationTime=update diagram  Latency=0  AutoFrameSizeCalculation=off
      link override Signal_Limit/_maxval: Value=KOUTP_LVDAFailinfo_flg_maxval
      link override Signal_Limit/_minval: Value=KOUTP_LVDAFailinfo_flg_minval
      link override Signal_Override/_ovrdflg: Value=KOUTP_LVDAFailinfo_flg_ovrdflg
      link override Signal_Override/_ovrdval: Value=KOUTP_LVDAFailinfo_flg_ovrdval
  VVMC_LVDAMuteSta_enum_Inproc : FVT_lib/outp/OverrideAndLimit  SystemSampleTime=-1  VariantActivationTime=update diagram  Latency=0  AutoFrameSizeCalculation=off
      link override Signal_Limit/_maxval: Value=KOUTP_LVDAMuteSta_enum_maxval
      link override Signal_Limit/_minval: Value=KOUTP_LVDAMuteSta_enum_minval
      link override Signal_Override/_ovrdflg: Value=KOUTP_LVDAMuteSta_enum_ovrdflg
      link override Signal_Override/_ovrdval: Value=KOUTP_LVDAMuteSta_enum_ovrdval
  VVMC_LVDAWarning_flg_Inproc : FVT_lib/outp/OverrideAndLimit  SystemSampleTime=-1  VariantActivationTime=update diagram  Latency=0  AutoFrameSizeCalculation=off
      link override Signal_Limit/_maxval: Value=KOUTP_LVDAWarning_flg_maxval
      link override Signal_Limit/_minval: Value=KOUTP_LVDAWarning_flg_minval
      link override Signal_Override/_ovrdflg: Value=KOUTP_LVDAWarning_flg_ovrdflg
      link override Signal_Override/_ovrdval: Value=KOUTP_LVDAWarning_flg_ovrdval
  VVMC_LatAccCtrl_flg_Inproc : FVT_lib/outp/OverrideAndLimit  SystemSampleTime=-1  VariantActivationTime=update diagram  Latency=0  AutoFrameSizeCalculation=off
      link override Signal_Limit/_maxval: Value=KOUTP_LatAccCtrl_flg_maxval
      link override Signal_Limit/_minval: Value=KOUTP_LatAccCtrl_flg_minval
      link override Signal_Override/_ovrdflg: Value=KOUTP_LatAccCtrl_flg_ovrdflg
      link override Signal_Override/_ovrdval: Value=KOUTP_LatAccCtrl_flg_ovrdval
  VVMC_LateralCtrl_flg_Inproc : FVT_lib/outp/OverrideAndLimit  SystemSampleTime=-1  VariantActivationTime=update diagram  Latency=0  AutoFrameSizeCalculation=off
      link override Signal_Limit/_maxval: Value=KOUTP_LateralCtrl_flg_maxval
      link override Signal_Limit/_minval: Value=KOUTP_LateralCtrl_flg_minval
      link override Signal_Override/_ovrdflg: Value=KOUTP_LateralCtrl_flg_ovrdflg
      link override Signal_Override/_ovrdval: Value=KOUTP_LateralCtrl_flg_ovrdval
  VVMC_LeftTurnLightReq_flg_Inproc : FVT_lib/outp/OverrideAndLimit  SystemSampleTime=-1  VariantActivationTime=update diagram  Latency=0  AutoFrameSizeCalculation=off
      link override Signal_Limit/_maxval: Value=KOUTP_LeftTurnLightReq_flg_maxval
      link override Signal_Limit/_minval: Value=KOUTP_LeftTurnLightReq_flg_minval
      link override Signal_Override/_ovrdflg: Value=KOUTP_LeftTurnLightReq_flg_ovrdflg
      link override Signal_Override/_ovrdval: Value=KOUTP_LeftTurnLightReq_flg_ovrdval
  VVMC_LimitPCT_pct_Inproc : FVT_lib/outp/OverrideAndLimit  SystemSampleTime=-1  VariantActivationTime=update diagram  Latency=0  AutoFrameSizeCalculation=off
      link override Signal_Limit/_maxval: Value=KOUTP_LimitPCT_pct_maxval
      link override Signal_Limit/_minval: Value=KOUTP_LimitPCT_pct_minval
      link override Signal_Override/_ovrdflg: Value=KOUTP_LimitPCT_pct_ovrdflg
      link override Signal_Override/_ovrdval: Value=KOUTP_LimitPCT_pct_ovrdval
  VVMC_LongAcc_Gps_Inproc : FVT_lib/outp/OverrideAndLimit  SystemSampleTime=-1  VariantActivationTime=update diagram  Latency=0  AutoFrameSizeCalculation=off
      link override Signal_Limit/_maxval: Value=KOUTP_LongAcc_Gps_maxval
      link override Signal_Limit/_minval: Value=KOUTP_LongAcc_Gps_minval
      link override Signal_Override/_ovrdflg: Value=KOUTP_LongAcc_Gps_ovrdflg
      link override Signal_Override/_ovrdval: Value=KOUTP_LongAcc_Gps_ovrdval
  VVMC_MSACtrlSta_enum_Inproc : FVT_lib/outp/OverrideAndLimit  SystemSampleTime=-1  VariantActivationTime=update diagram  Latency=0  AutoFrameSizeCalculation=off
      link override Signal_Limit/_maxval: Value=KOUTP_MSACtrlSta_enum_maxval
      link override Signal_Limit/_minval: Value=KOUTP_MSACtrlSta_enum_minval
      link override Signal_Override/_ovrdflg: Value=KOUTP_MSACtrlSta_enum_ovrdflg
      link override Signal_Override/_ovrdval: Value=KOUTP_MSACtrlSta_enum_ovrdval
  VVMC_MeterIndSpeed_raw32_Inproc : FVT_lib/outp/OverrideAndLimit  SystemSampleTime=-1  VariantActivationTime=update diagram  Latency=0  AutoFrameSizeCalculation=off
      link override Signal_Limit/_maxval: Value=KOUTP_MeterIndSpeed_raw32_maxval
      link override Signal_Limit/_minval: Value=KOUTP_MeterIndSpeed_raw32_minval
      link override Signal_Override/_ovrdflg: Value=KOUTP_MeterIndSpeed_raw32_ovrdflg
      link override Signal_Override/_ovrdval: Value=KOUTP_MeterIndSpeed_raw32_ovrdval
  VVMC_RearWhlSlipRatioCtrl_flg_Inproc : FVT_lib/outp/OverrideAndLimit  SystemSampleTime=-1  VariantActivationTime=update diagram  Latency=0  AutoFrameSizeCalculation=off
      link override Signal_Limit/_maxval: Value=KOUTP_RearWhlSlipRatioCtrl_flg_maxval
      link override Signal_Limit/_minval: Value=KOUTP_RearWhlSlipRatioCtrl_flg_minval
      link override Signal_Override/_ovrdflg: Value=KOUTP_RearWhlSlipRatioCtrl_flg_ovrdflg
      link override Signal_Override/_ovrdval: Value=KOUTP_RearWhlSlipRatioCtrl_flg_ovrdval
  VVMC_RightTurnLightReq_flg_Inproc : FVT_lib/outp/OverrideAndLimit  SystemSampleTime=-1  VariantActivationTime=update diagram  Latency=0  AutoFrameSizeCalculation=off
      link override Signal_Limit/_maxval: Value=KOUTP_RightTurnLightReq_flg_maxval
      link override Signal_Limit/_minval: Value=KOUTP_RightTurnLightReq_flg_minval
      link override Signal_Override/_ovrdflg: Value=KOUTP_RightTurnLightReq_flg_ovrdflg
      link override Signal_Override/_ovrdval: Value=KOUTP_RightTurnLightReq_flg_ovrdval
  VVMC_SPD2ACCAct_flg_Inproc : FVT_lib/outp/OverrideAndLimit  SystemSampleTime=-1  VariantActivationTime=update diagram  Latency=0  AutoFrameSizeCalculation=off
      link override Signal_Limit/_maxval: Value=KOUTP_SPD2ACCAct_flg_maxval
      link override Signal_Limit/_minval: Value=KOUTP_SPD2ACCAct_flg_minval
      link override Signal_Override/_ovrdflg: Value=KOUTP_SPD2ACCAct_flg_ovrdflg
      link override Signal_Override/_ovrdval: Value=KOUTP_SPD2ACCAct_flg_ovrdval
  VVMC_SafetyCtrl_flg_Inproc : FVT_lib/outp/OverrideAndLimit  SystemSampleTime=-1  VariantActivationTime=update diagram  Latency=0  AutoFrameSizeCalculation=off
      link override Signal_Limit/_maxval: Value=KOUTP_SafetyCtrl_flg_maxval
      link override Signal_Limit/_minval: Value=KOUTP_SafetyCtrl_flg_minval
      link override Signal_Override/_ovrdflg: Value=KOUTP_SafetyCtrl_flg_ovrdflg
      link override Signal_Override/_ovrdval: Value=KOUTP_SafetyCtrl_flg_ovrdval
  VVMC_SingleWhlSlipRatioCtrl_flg_Inproc : FVT_lib/outp/OverrideAndLimit  SystemSampleTime=-1  VariantActivationTime=update diagram  Latency=0  AutoFrameSizeCalculation=off
      link override Signal_Limit/_maxval: Value=KOUTP_SingleWhlSlipRatioCtrl_flg_maxval
      link override Signal_Limit/_minval: Value=KOUTP_SingleWhlSlipRatioCtrl_flg_minval
      link override Signal_Override/_ovrdflg: Value=KOUTP_SingleWhlSlipRatioCtrl_flg_ovrdflg
      link override Signal_Override/_ovrdval: Value=KOUTP_SingleWhlSlipRatioCtrl_flg_ovrdval
  VVMC_TargetType_enum_Inproc : FVT_lib/outp/OverrideAndLimit  SystemSampleTime=-1  VariantActivationTime=update diagram  Latency=0  AutoFrameSizeCalculation=off
      link override Signal_Limit/_maxval: Value=KOUTP_TargetType_enum_maxval
      link override Signal_Limit/_minval: Value=KOUTP_TargetType_enum_minval
      link override Signal_Override/_ovrdflg: Value=KOUTP_TargetType_enum_ovrdflg
      link override Signal_Override/_ovrdval: Value=KOUTP_TargetType_enum_ovrdval
  VVMC_TimeGapCalcu_s_Inproc : FVT_lib/outp/OverrideAndLimit  SystemSampleTime=-1  VariantActivationTime=update diagram  Latency=0  AutoFrameSizeCalculation=off
      link override Signal_Limit/_maxval: Value=KOUTP_TimeGapCalcu_s_maxval
      link override Signal_Limit/_minval: Value=KOUTP_TimeGapCalcu_s_minval
      link override Signal_Override/_ovrdflg: Value=KOUTP_TimeGapCalcu_s_ovrdflg
      link override Signal_Override/_ovrdval: Value=KOUTP_TimeGapCalcu_s_ovrdval
  VVMC_TimeGapLevel_enum_Inproc : FVT_lib/outp/OverrideAndLimit  SystemSampleTime=-1  VariantActivationTime=update diagram  Latency=0  AutoFrameSizeCalculation=off
      link override Signal_Limit/_maxval: Value=KOUTP_TimeGapLevel_enum_maxval
      link override Signal_Limit/_minval: Value=KOUTP_TimeGapLevel_enum_minval
      link override Signal_Override/_ovrdflg: Value=KOUTP_TimeGapLevel_enum_ovrdflg
      link override Signal_Override/_ovrdval: Value=KOUTP_TimeGapLevel_enum_ovrdval
  VVMC_VMCACCCtrlAvail_flg_Inproc : FVT_lib/outp/OverrideAndLimit  SystemSampleTime=-1  VariantActivationTime=update diagram  Latency=0  AutoFrameSizeCalculation=off
      link override Signal_Limit/_maxval: Value=KOUTP_VMCACCCtrlAvail_flg_maxval
      link override Signal_Limit/_minval: Value=KOUTP_VMCACCCtrlAvail_flg_minval
      link override Signal_Override/_ovrdflg: Value=KOUTP_VMCACCCtrlAvail_flg_ovrdflg
      link override Signal_Override/_ovrdval: Value=KOUTP_VMCACCCtrlAvail_flg_ovrdval
  VVMC_VMCAEBCtrlAvail_flg_Inproc : FVT_lib/outp/OverrideAndLimit  SystemSampleTime=-1  VariantActivationTime=update diagram  Latency=0  AutoFrameSizeCalculation=off
      link override Signal_Limit/_maxval: Value=KOUTP_VMCAEBCtrlAvail_flg_maxval
      link override Signal_Limit/_minval: Value=KOUTP_VMCAEBCtrlAvail_flg_minval
      link override Signal_Override/_ovrdflg: Value=KOUTP_VMCAEBCtrlAvail_flg_ovrdflg
      link override Signal_Override/_ovrdval: Value=KOUTP_VMCAEBCtrlAvail_flg_ovrdval
  VVMC_VMCCCCtrlAvail_flg_Inproc : FVT_lib/outp/OverrideAndLimit  SystemSampleTime=-1  VariantActivationTime=update diagram  Latency=0  AutoFrameSizeCalculation=off
      link override Signal_Limit/_maxval: Value=KOUTP_VMCCCCtrlAvail_flg_maxval
      link override Signal_Limit/_minval: Value=KOUTP_VMCCCCtrlAvail_flg_minval
      link override Signal_Override/_ovrdflg: Value=KOUTP_VMCCCCtrlAvail_flg_ovrdflg
      link override Signal_Override/_ovrdval: Value=KOUTP_VMCCCCtrlAvail_flg_ovrdval
  VVMC_VMCMSACtrlAvail_flg_Inproc : FVT_lib/outp/OverrideAndLimit  SystemSampleTime=-1  VariantActivationTime=update diagram  Latency=0  AutoFrameSizeCalculation=off
      link override Signal_Limit/_maxval: Value=KOUTP_VMCMSACtrlAvail_flg_maxval
      link override Signal_Limit/_minval: Value=KOUTP_VMCMSACtrlAvail_flg_minval
      link override Signal_Override/_ovrdflg: Value=KOUTP_VMCMSACtrlAvail_flg_ovrdflg
      link override Signal_Override/_ovrdval: Value=KOUTP_VMCMSACtrlAvail_flg_ovrdval
  VVMC_VehicleSpeed_kph_Inproc : FVT_lib/outp/OverrideAndLimit  SystemSampleTime=-1  VariantActivationTime=update diagram  Latency=0  AutoFrameSizeCalculation=off
      link override Signal_Limit/_maxval: Value=KOUTP_VehicleSpeed_kph_maxval
      link override Signal_Limit/_minval: Value=KOUTP_VehicleSpeed_kph_minval
      link override Signal_Override/_ovrdflg: Value=KOUTP_VehicleSpeed_kph_ovrdflg
      link override Signal_Override/_ovrdval: Value=KOUTP_VehicleSpeed_kph_ovrdval
  VVMC_VehicleSpeed_mph_Inproc : FVT_lib/outp/OverrideAndLimit  SystemSampleTime=-1  VariantActivationTime=update diagram  Latency=0  AutoFrameSizeCalculation=off
      link override Signal_Limit/_maxval: Value=KOUTP_VehicleSpeed_mph_maxval
      link override Signal_Limit/_minval: Value=KOUTP_VehicleSpeed_mph_minval
      link override Signal_Override/_ovrdflg: Value=KOUTP_VehicleSpeed_mph_ovrdflg
      link override Signal_Override/_ovrdval: Value=KOUTP_VehicleSpeed_mph_ovrdval
  VOUTP_EACEnDemand_enum : Outport
  VOUTP_CACTempOverHigh_flg : Outport  Port=2
  VOUTP_CACPresWarn_flg : Outport  Port=3
  VOUTP_CACPresReady_flg : Outport  Port=4
  VOUTP_EHPSEnDemand_enum : Outport  Port=5
  VOUTP_CACOverrun_flg : Outport  Port=6
  VOUTP_CACRunFail_flg : Outport  Port=7
  VOUTP_CACFanReq_flg : Outport  Port=8
  VOUTP_EHPSMotorDemSpd_rpm : Outport  Port=9
  VOUTP_EHPSSpdDemTimeout_flg : Outport  Port=10
  VOUTP_EHPSEnTimeout_flg : Outport  Port=11
  VOUTP_EHPSDisEnTimeout_flg : Outport  Port=12
  VOUTP_DCDCEnDemamd_enum : Outport  Port=13
  VOUTP_EHPSSpdCtrlMode_enum : Outport  Port=14
  VOUTP_EACSpdDemand_rpm : Outport  Port=15
  VOUTP_VehSpeed_kph : Outport  Port=16
  VOUTP_VehSpeedTimeOut_flg : Outport  Port=17
  VOUTP_FSOffSw_enum : Outport  Port=18
  VOUTP_FSOffSwTimeOut_flg : Outport  Port=19
  VOUTP_ChrgPlugSta_enum : Outport  Port=20
  VOUTP_PASDRMR_cm : Outport  Port=21
  VOUTP_PASDRML_cm : Outport  Port=22
  VOUTP_PASDRCR_cm : Outport  Port=23
  VOUTP_PASDRCL_cm : Outport  Port=24
  VOUTP_PASDFMR_cm : Outport  Port=25
  VOUTP_PASDFML_cm : Outport  Port=26
  VOUTP_PASDFCR_cm : Outport  Port=27
  VOUTP_PASDFCL_cm : Outport  Port=28
  VOUTP_APSDRLR_cm : Outport  Port=29
  VOUTP_APSDRLL_cm : Outport  Port=30
  VOUTP_APSDFLR_cm : Outport  Port=31
  VOUTP_APSDFLL_cm : Outport  Port=32
  VOUTP_PASAFCL_enum : Outport  Port=33
  VOUTP_PASARMR_enum : Outport  Port=34
  VOUTP_PASARML_enum : Outport  Port=35
  VOUTP_PASARCR_enum : Outport  Port=36
  VOUTP_PASARCL_enum : Outport  Port=37
  VOUTP_PASAFMR_enum : Outport  Port=38
  VOUTP_PASAFML_enum : Outport  Port=39
  VOUTP_PASAFCR_enum : Outport  Port=40
  VOUTP_USSStaRMR_flg : Outport  Port=41
  VOUTP_USSStaRML_flg : Outport  Port=42
  VOUTP_USSStaRLR_flg : Outport  Port=43
  VOUTP_USSStaRLL_flg : Outport  Port=44
  VOUTP_USSStaRCR_flg : Outport  Port=45
  VOUTP_USSStaRCL_flg : Outport  Port=46
  VOUTP_USSStaFMR_flg : Outport  Port=47
  VOUTP_USSStaFML_flg : Outport  Port=48
  VOUTP_USSStaFLR_flg : Outport  Port=49
  VOUTP_USSStaFLL_flg : Outport  Port=50
  VOUTP_USSStaFCR_flg : Outport  Port=51
  VOUTP_USSStaFCL_flg : Outport  Port=52
  VOUTP_Chime_enum : Outport  Port=53
  VOUTP_SNSRLayout_enum : Outport  Port=54
  VOUTP_StaFSya_flg : Outport  Port=55
  VOUTP_ModOperation_enum : Outport  Port=56
  VOUTP_BrkPedalPos_pct : Outport  Port=57
  VOUTP_BrkPedalPosTimeOut_flg : Outport  Port=58
  VOUTP_LFRawWhlSpeed_kph : Outport  Port=59
  VOUTP_LFRawWhlSpeedTimeOut_flg : Outport  Port=60
  VOUTP_RFRawWhlSpeed_kph : Outport  Port=61
  VOUTP_RFRawWhlSpeedTimeOut_flg : Outport  Port=62
  VOUTP_LRRawWhlSpeed_kph : Outport  Port=63
  VOUTP_LRRawWhlSpeedTimeOut_flg : Outport  Port=64
  VOUTP_RRRawWhlSpeed_kph : Outport  Port=65
  VOUTP_RRRawWhlSpeedTimeOut_flg : Outport  Port=66
  VOUTP_LFRawWhlSpeedV_flg : Outport  Port=67
  VOUTP_LFRawWhlSpeedVTimeOut_flg : Outport  Port=68
  VOUTP_RFRawWhlSpeedV_flg : Outport  Port=69
  VOUTP_RFRawWhlSpeedVTimeOut_flg : Outport  Port=70
  VOUTP_LRRawWhlSpeedV_flg : Outport  Port=71
  VOUTP_LRRawWhlSpeedVTimeOut_flg : Outport  Port=72
  VOUTP_RRRawWhlSpeedV_flg : Outport  Port=73
  VOUTP_RRRawWhlSpeedVTimeOut_flg : Outport  Port=74
  VOUTP_LFWhlRotDir_enum : Outport  Port=75
  VOUTP_LFWhlRotDirTimeOut_flg : Outport  Port=76
  VOUTP_RFWhlRotDir_enum : Outport  Port=77
  VOUTP_RFWhlRotDirTimeOut_flg : Outport  Port=78
  VOUTP_LRWhlRotDir_enum : Outport  Port=79
  VOUTP_LRWhlRotDirTimeOut_flg : Outport  Port=80
  VOUTP_RRWhlRotDir_enum : Outport  Port=81
  VOUTP_RRWhlRotDirTimeOut_flg : Outport  Port=82
  VOUTP_LFPulseCountV_flg : Outport  Port=83
  VOUTP_LFPulseCountVTimeOut_flg : Outport  Port=84
  VOUTP_RFPulseCountV_flg : Outport  Port=85
  VOUTP_RFPulseCountVTimeOut_flg : Outport  Port=86
  VOUTP_LRPulseCountV_flg : Outport  Port=87
  VOUTP_LRPulseCountVTimeOut_flg : Outport  Port=88
  VOUTP_RRPulseCountV_flg : Outport  Port=89
  VOUTP_RRPulseCountVTimeOut_flg : Outport  Port=90
  VOUTP_LFPulseCount_enum : Outport  Port=91
  VOUTP_LFPulseCountTimeOut_flg : Outport  Port=92
  VOUTP_RFPulseCount_enum : Outport  Port=93
  VOUTP_RFPulseCountTimeOut_flg : Outport  Port=94
  VOUTP_LRPulseCount_enum : Outport  Port=95
  VOUTP_LRPulseCountTimeOut_flg : Outport  Port=96
  VOUTP_RRPulseCount_enum : Outport  Port=97
  VOUTP_RRPulseCountTimeOut_flg : Outport  Port=98
  VOUTP_ShifterHandleCmd_enum : Outport  Port=99
  VOUTP_ShifterHandleCmdTimeOut_flg : Outport  Port=100
  VOUTP_DriIntend_enum : Outport  Port=101
  VOUTP_DriIntendTimeOut_flg : Outport  Port=102
  VOUTP_EPSAOIControl_enum : Outport  Port=103
  VOUTP_EPSAOIControlTimeOut_flg : Outport  Port=104
  VOUTP_SASAngle_Deg : Outport  Port=105
  VOUTP_SASAngleTimeOut_flg : Outport  Port=106
  VOUTP_SASSpeed_degps : Outport  Port=107
  VOUTP_SASSpeedTimeOut_flg : Outport  Port=108
  VOUTP_SASSpeedValid_flg : Outport  Port=109
  VOUTP_SASSpeedValidTimeOut_flg : Outport  Port=110
  VOUTP_SASCAL_flg : Outport  Port=111
  VOUTP_SASCALTimeOut_flg : Outport  Port=112
  VOUTP_SASV_flg : Outport  Port=113
  VOUTP_SASVTimeOut_flg : Outport  Port=114
  VOUTP_GRADE_Deg : Outport  Port=115
  VOUTP_GRADETimeOut_flg : Outport  Port=116
  VOUTP_YawRate_degps : Outport  Port=117
  VOUTP_YawRateTimeOut_flg : Outport  Port=118
  VOUTP_LatAccel_Gps : Outport  Port=119
  VOUTP_LatAccelTimeOut_flg : Outport  Port=120
  VOUTP_LongAccel_Gps : Outport  Port=121
  VOUTP_LongAccelTimeOut_flg : Outport  Port=122
  VOUTP_MCPressure_bar : Outport  Port=123
  VOUTP_MCPressureTimeOut_flg : Outport  Port=124
  VOUTP_YawRateV_flg : Outport  Port=125
  VOUTP_YawRateVTimeOut_flg : Outport  Port=126
  VOUTP_LatAccelV_flg : Outport  Port=127
  VOUTP_LatAccelVTimeOut_flg : Outport  Port=128
  VOUTP_LongAccelV_flg : Outport  Port=129
  VOUTP_LongAccelVTimeOut_flg : Outport  Port=130
  VOUTP_MCPressureV_bar : Outport  Port=131
  VOUTP_MCPressureVTimeOut_flg : Outport  Port=132
  VOUTP_BrkSwSta_flg : Outport  Port=133
  VOUTP_BrkSwStaTimeOut_flg : Outport  Port=134
  VOUTP_BrkSwV_flg : Outport  Port=135
  VOUTP_BrkSwVTimeOut_flg : Outport  Port=136
  VOUTP_ESCStandstill_flg : Outport  Port=137
  VOUTP_ESCStandstillTimeOut_flg : Outport  Port=138
  VOUTP_ESCAPSSta_enum : Outport  Port=139
  VOUTP_ESCAPSStaTimeOut_flg : Outport  Port=140
  VOUTP_EPBExtReleaseAvail_flg : Outport  Port=141
  VOUTP_EPBExtReleaseAvailTimeOut_flg : Outport  Port=142
  VOUTP_EPBExtApplyAvail_flg : Outport  Port=143
  VOUTP_EPBExtApplyAvailTimeOut_flg : Outport  Port=144
  VOUTP_EPBErrSta_enum : Outport  Port=145
  VOUTP_EPBErrStaTimeOut_flg : Outport  Port=146
  VOUTP_EPBSta_enum : Outport  Port=147
  VOUTP_EPBStaTimeOut_flg : Outport  Port=148
  VOUTP_AVMparkingcancel_enum : Outport  Port=149
  VOUTP_AVMparkingcancelTimeOut_flg : Outport  Port=150
  VOUTP_AVMparkingexcute_enum : Outport  Port=151
  VOUTP_AVMparkingexcuteTimeOut_flg : Outport  Port=152
  VOUTP_AVMParkingmode_enum : Outport  Port=153
  VOUTP_AVMParkingmodeTimeOut_flg : Outport  Port=154
  VOUTP_AVMErrSTA_flg : Outport  Port=155
  VOUTP_AVMErrSTATimeOut_flg : Outport  Port=156
  VOUTP_IVIStatus_flg : Outport  Port=157
  VOUTP_IVIStatusTimeOut_flg : Outport  Port=158
  VOUTP_CAASSw_enum : Outport  Port=159
  VOUTP_CAASSwTimeOut_flg : Outport  Port=160
  VOUTP_IVIScreen_enum : Outport  Port=161
  VOUTP_IVIScreenTimeOut_flg : Outport  Port=162
  VOUTP_ABSActive_flg : Outport  Port=163
  VOUTP_ABSActiveTimeOut_flg : Outport  Port=164
  VOUTP_TCSActive_flg : Outport  Port=165
  VOUTP_TCSActiveTimeOut_flg : Outport  Port=166
  VOUTP_DriverSeatBeltCmd_flg : Outport  Port=167
  VOUTP_DriverSeatBeltCmdTimeOut_flg : Outport  Port=168
  VOUTP_APSProgressPCT_pct : Outport  Port=169
  VOUTP_APSRQDisplay_enum : Outport  Port=170
  VOUTP_APSSWVer_enum : Outport  Port=171
  VOUTP_APSHWVer_enum : Outport  Port=172
  VOUTP_APSExitCondition_enum : Outport  Port=173
  VOUTP_APSAngleTarget_Deg : Outport  Port=174
  VOUTP_APSVRqEPASCtrl_flg : Outport  Port=175
  VOUTP_APSRqEPASCtrl_flg : Outport  Port=176
  VOUTP_CAASSta_enum : Outport  Port=177
  VOUTP_DKCPDkeyAreaRAPSSta_enum : Outport  Port=178
  VOUTP_DKCParkingModeCmd_enum : Outport  Port=179
  VOUTP_PUIDLowPower_flg : Outport  Port=180
  VOUTP_CAASVMCReqA_flg : Outport  Port=181
  VOUTP_APSShiftPosnReq_enum : Outport  Port=182
  VOUTP_APSSpeedCMD_kph : Outport  Port=183
  VOUTP_APSVMCReqA_flg : Outport  Port=184
  VOUTP_RAPSBCMLamp_enum : Outport  Port=185
  VOUTP_RAPSBCMLockReq_flg : Outport  Port=186
  VOUTP_APSPwrReq_enum : Outport  Port=187
  VOUTP_RAPSErrWarnSta_enum : Outport  Port=188
  VOUTP_RAPSErrLv1_flg : Outport  Port=189
  VOUTP_IVIUserTakeOverAPSSta_flg : Outport  Port=190
  VOUTP_FDCBCMLBeamCmd_flg : Outport  Port=191
  VOUTP_FDCBCMPLampCmd_flg : Outport  Port=192
  VOUTP_FDCBCMHBeamCmd_flg : Outport  Port=193
  VOUTP_FDCBCMSMKLCmd_flg : Outport  Port=194
  VOUTP_FDCBCMSMKRCmd_flg : Outport  Port=195
  VOUTP_FDCBCMDVRSignalLCmd_flg : Outport  Port=196
  VOUTP_FDCBCMDVRSignalRCmd_flg : Outport  Port=197
  VOUTP_FDCBCMBSDBuzzerCmd_flg : Outport  Port=198
  VOUTP_FDCBCMSLTLpCmd_flg : Outport  Port=199
  VOUTP_FDCBCMSRTLpCmd_flg : Outport  Port=200
  VOUTP_FDCBCMLTurnLpCmd_flg : Outport  Port=201
  VOUTP_FDCBCMRTurnLpCmd_flg : Outport  Port=202
  VOUTP_FDCBCMStopINDCmd_flg : Outport  Port=203
  VOUTP_FDCBCMSTOPBALLCmd_flg : Outport  Port=204
  VOUTP_FDCBCMInnerCallBellCmd_flg : Outport  Port=205
  VOUTP_FDCBCMCallBellCmd_flg : Outport  Port=206
  VOUTP_FDCBCMWiperHCmd_flg : Outport  Port=207
  VOUTP_FDCBCMWasherCmd_flg : Outport  Port=208
  VOUTP_FDCBCMWiperLCmd_flg : Outport  Port=209
  VOUTP_FDCBCMLDRLCmd_flg : Outport  Port=210
  VOUTP_FDCBCMRDRLCmd_flg : Outport  Port=211
  VOUTP_FDCBCMRFLampCmd_flg : Outport  Port=212
  VOUTP_TurnLpPatternSta_enum : Outport  Port=213
  VOUTP_FDCBCMFDoorSta_flg : Outport  Port=214
  VOUTP_FDCBCMMDoorSta_flg : Outport  Port=215
  VOUTP_FDCBCMRDoorSta_flg : Outport  Port=216
  VOUTP_FDCBCMRoomLpAmbCmd_flg : Outport  Port=217
  VOUTP_FDCBCMLBSDRCmd_flg : Outport  Port=218
  VOUTP_FDCBCMLBSDYCmd_flg : Outport  Port=219
  VOUTP_FDCBCMRBSDRCmd_flg : Outport  Port=220
  VOUTP_FDCBCMRBSDYCmd_flg : Outport  Port=221
  VOUTP_FDCBCMEmExitSWSta_flg : Outport  Port=222
  VOUTP_InnerBuzzerModeSta_enum : Outport  Port=223
  VOUTP_FDCBCMInnerBuzzerCmd_flg : Outport  Port=224
  VOUTP_FDCBCMRoomLpAmbSetSta_flg : Outport  Port=225
  VOUTP_FDCBCMRoomLpSetSta_flg : Outport  Port=226
  VOUTP_FDCBCMFRoomLpSetSta_pct : Outport  Port=227
  VOUTP_FDCBCMFRoomLpCmd_pct : Outport  Port=228
  VOUTP_FDCBCMMRoomLpSetSta_pct : Outport  Port=229
  VOUTP_FDCBCMMRoomLpCmd_pct : Outport  Port=230
  VOUTP_FDCBCMRRoomLpSetSta_pct : Outport  Port=231
  VOUTP_FDCBCMRRoomLpCmd_pct : Outport  Port=232
  VOUTP_FDCBCMHelpINDCmd_flg : Outport  Port=233
  VOUTP_FDCBCMOSDrOpenSWSta_enum : Outport  Port=234
  VOUTP_FDCBCMEmSVCmd_flg : Outport  Port=235
  VOUTP_FDCBCMFDOpenSVCmd_flg : Outport  Port=236
  VOUTP_FDCBCMFDCloseSVCmd_flg : Outport  Port=237
  VOUTP_FDCBCMMDOpenSVCmd_flg : Outport  Port=238
  VOUTP_FDCBCMMDCloseSVCmd_flg : Outport  Port=239
  VOUTP_FDCBCMLTurnSWSta_flg : Outport  Port=240
  VOUTP_FDCBCMRTurnSWSta_flg : Outport  Port=241
  VOUTP_FDCBCMRGearSta_flg : Outport  Port=242
  VOUTP_FDCBCMBrakeCmd_flg : Outport  Port=243
  VOUTP_FDCBCMTurnBuzzerENSta_flg : Outport  Port=244
  VOUTP_WakeUp_flg : Outport  Port=245
  VOUTP_KeepWakeUp_flg : Outport  Port=246
  VOUTP_C3BMS6RCDTC_raw32 : Outport  Port=247
  VOUTP_C3BMS6CSDTC_raw32 : Outport  Port=248
  VOUTP_C3BMS6LCDTC_raw32 : Outport  Port=249
  VOUTP_C3BMS1RCDTC_raw32 : Outport  Port=250
  VOUTP_C3BMS1CSDTC_raw32 : Outport  Port=251
  VOUTP_C3BMS1LCDTC_raw32 : Outport  Port=252
  VOUTP_C3CCU1RCDTC_raw32 : Outport  Port=253
  VOUTP_C3CCU1CSDTC_raw32 : Outport  Port=254
  VOUTP_C3CCU1LCDTC_raw32 : Outport  Port=255
  VOUTP_C3CCU2RCDTC_raw32 : Outport  Port=256
  VOUTP_C3CCU2CSDTC_raw32 : Outport  Port=257
  VOUTP_C3CCU2LCDTC_raw32 : Outport  Port=258
  VOUTP_C1ABM1RCDTC_raw32 : Outport  Port=259
  VOUTP_C1ABM1CSDTC_raw32 : Outport  Port=260
  VOUTP_C1ABM1LCDTC_raw32 : Outport  Port=261
  VOUTP_Lv1ErrDTC_raw32 : Outport  Port=262
  VOUTP_Lv2ErrDTC_raw32 : Outport  Port=263
  VOUTP_Lv3ErrDTC_raw32 : Outport  Port=264
  VOUTP_Lv4ErrDTC_raw32 : Outport  Port=265
  VOUTP_BrkSWErrDTC_raw32 : Outport  Port=266
  VOUTP_BrkSWNoBacDTC_raw32 : Outport  Port=267
  VOUTP_KeyAuthDTC_raw32 : Outport  Port=268
  VOUTP_ONtoRdyDTC_raw32 : Outport  Port=269
  VOUTP_HVB4PreDTC_raw32 : Outport  Port=270
  VOUTP_MCU4PreDTC_raw32 : Outport  Port=271
  VOUTP_DCDC4PreDTC_raw32 : Outport  Port=272
  VOUTP_HVRlyCloDTC_raw32 : Outport  Port=273
  VOUTP_BMSRdyDTC_raw32 : Outport  Port=274
  VOUTP_DCDCEnaDTC_raw32 : Outport  Port=275
  VOUTP_HiLvSaChkDTC_raw32 : Outport  Port=276
  VOUTP_MidLvSaChkDTC_raw32 : Outport  Port=277
  VOUTP_MCUDisDTC_raw32 : Outport  Port=278
  VOUTP_DCDCDisDTC_raw32 : Outport  Port=279
  VOUTP_HVRlyOpDTC_raw32 : Outport  Port=280
  VOUTP_MCUActDTC_raw32 : Outport  Port=281
  VOUTP_OBC4PreDTC_raw32 : Outport  Port=282
  VOUTP_IniLVLoDTC_raw32 : Outport  Port=283
  VOUTP_LVSupLoDTC_raw32 : Outport  Port=284
  VOUTP_LVSupHiDTC_raw32 : Outport  Port=285
  VOUTP_DrStSWDTC_raw32 : Outport  Port=286
  VOUTP_FLDoorSWDTC_raw32 : Outport  Port=287
  VOUTP_RLDoorSWDTC_raw32 : Outport  Port=288
  VOUTP_FRDoorSWDTC_raw32 : Outport  Port=289
  VOUTP_RRDoorSWDTC_raw32 : Outport  Port=290
  VOUTP_HoodSWDTC_raw32 : Outport  Port=291
  VOUTP_TailgaSWDTC_raw32 : Outport  Port=292
  VOUTP_EDriveSysErrVCUErr_flg : Outport  Port=293
  VOUTP_VehMalfunLevel_enum : Outport  Port=294
  VOUTP_APS1SigOoRDTC_raw32 : Outport  Port=295
  VOUTP_APS2SigOoRDTC_raw32 : Outport  Port=296
  VOUTP_APSCorrErrDTC_raw32 : Outport  Port=297
  VOUTP_MCUF1NoComDTC_raw32 : Outport  Port=298
  VOUTP_MCUR1NoComDTC_raw32 : Outport  Port=299
  VOUTP_Shifter1NoComDTC_raw32 : Outport  Port=300
  VOUTP_ESC7NoComDTC_raw32 : Outport  Port=301
  VOUTP_ESC1NoComDTC_raw32 : Outport  Port=302
  VOUTP_ESC5NoComDTC_raw32 : Outport  Port=303
  VOUTP_EnterNewOperCyc_flg : Outport  Port=304
  VOUTP_DiagHCrashDTC_raw32 : Outport  Port=305
  VOUTP_DiagFLTSDTC_raw32 : Outport  Port=306
  VOUTP_DiagFRTSDTC_raw32 : Outport  Port=307
  VOUTP_DiagRLTSDTC_raw32 : Outport  Port=308
  VOUTP_DiagRRTSDTC_raw32 : Outport  Port=309
  VOUTP_FCLUSSDTC_raw32 : Outport  Port=310
  VOUTP_FMLUSSDTC_raw32 : Outport  Port=311
  VOUTP_FMRUSSDTC_raw32 : Outport  Port=312
  VOUTP_FCRUSSDTC_raw32 : Outport  Port=313
  VOUTP_RCLUSSDTC_raw32 : Outport  Port=314
  VOUTP_RMLUSSDTC_raw32 : Outport  Port=315
  VOUTP_RMRUSSDTC_raw32 : Outport  Port=316
  VOUTP_RCRUSSDTC_raw32 : Outport  Port=317
  VOUTP_FLLUSSDTC_raw32 : Outport  Port=318
  VOUTP_FLRUSSDTC_raw32 : Outport  Port=319
  VOUTP_RLLUSSDTC_raw32 : Outport  Port=320
  VOUTP_RLRUSSDTC_raw32 : Outport  Port=321
  VOUTP_FCM2NoComDTC_raw32 : Outport  Port=322
  VOUTP_FCM2RCErrDTC_raw32 : Outport  Port=323
  VOUTP_FCM2CSErrDTC_raw32 : Outport  Port=324
  VOUTP_FCM3NoComDTC_raw32 : Outport  Port=325
  VOUTP_FCM3RCErrDTC_raw32 : Outport  Port=326
  VOUTP_FCM3CSErrDTC_raw32 : Outport  Port=327
  VOUTP_FCM4NoComDTC_raw32 : Outport  Port=328
  VOUTP_FCM4CSErrDTC_raw32 : Outport  Port=329
  VOUTP_FCM5NoComDTC_raw32 : Outport  Port=330
  VOUTP_FCM5CSErrDTC_raw32 : Outport  Port=331
  VOUTP_ZoneSCPNoComDTC_raw32 : Outport  Port=332
  VOUTP_BMSSigErrDetDTC_raw32 : Outport  Port=333
  VOUTP_FCMACCSigErrDetDTC_raw32 : Outport  Port=334
  VOUTP_FrMCUSigErrDetDTC_raw32 : Outport  Port=335
  VOUTP_RrMCUSigErrDetDTC_raw32 : Outport  Port=336
  VOUTP_CCUSigErrDetDTC_raw32 : Outport  Port=337
  VOUTP_ACCAccelCmdErrDetDTC_raw32 : Outport  Port=338
  VOUTP_ACCMalfuncDetDTC_raw32 : Outport  Port=339
  VOUTP_CCMalfuncDetDTC_raw32 : Outport  Port=340
  VOUTP_MSAMalfuncDetDTC_raw32 : Outport  Port=341
  VOUTP_ISAMalfuncDetDTC_raw32 : Outport  Port=342
  VOUTP_MCUF1RCErrDTC_raw32 : Outport  Port=343
  VOUTP_MCUR1RCErrDTC_raw32 : Outport  Port=344
  VOUTP_MCUF1CSErrDTC_raw32 : Outport  Port=345
  VOUTP_MCUR1CSErrDTC_raw32 : Outport  Port=346
  VOUTP_Shifter1RCErrDTC_raw32 : Outport  Port=347
  VOUTP_Shifter1CSErrDTC_raw32 : Outport  Port=348
  VOUTP_ESC7RCErrDTC_raw32 : Outport  Port=349
  VOUTP_ESC7CSErrDTC_raw32 : Outport  Port=350
  VOUTP_ESC1RCErrDTC_raw32 : Outport  Port=351
  VOUTP_ESC1CSErrDTC_raw32 : Outport  Port=352
  VOUTP_ESC5RCErrDTC_raw32 : Outport  Port=353
  VOUTP_ESC5CSErrDTC_raw32 : Outport  Port=354
  VOUTP_FrMCUTqErrDTC_raw32 : Outport  Port=355
  VOUTP_RrMCUTqErrDTC_raw32 : Outport  Port=356
  VOUTP_LFBatwarnDTC_raw32 : Outport  Port=357
  VOUTP_RFBatwarnDTC_raw32 : Outport  Port=358
  VOUTP_LRBatwarnDTC_raw32 : Outport  Port=359
  VOUTP_RRBatwarnDTC_raw32 : Outport  Port=360
  VOUTP_LFPressIndiDTC_raw32 : Outport  Port=361
  VOUTP_RFPressIndiDTC_raw32 : Outport  Port=362
  VOUTP_LRPressIndiDTC_raw32 : Outport  Port=363
  VOUTP_RRPressIndiDTC_raw32 : Outport  Port=364
  VOUTP_LFWheelTmpHighDTC_raw32 : Outport  Port=365
  VOUTP_RFWheelTmpHighDTC_raw32 : Outport  Port=366
  VOUTP_LRWheelTmpHighDTC_raw32 : Outport  Port=367
  VOUTP_RRWheelTmpHighDTC_raw32 : Outport  Port=368
  VOUTP_LFSensorFailDTC_raw32 : Outport  Port=369
  VOUTP_RFSensorFailDTC_raw32 : Outport  Port=370
  VOUTP_LRSensorFailDTC_raw32 : Outport  Port=371
  VOUTP_RRSensorFailDTC_raw32 : Outport  Port=372
  VOUTP_C1EPAS2LCDTC_raw32 : Outport  Port=373
  VOUTP_5vAPS1PwrErrDTC_raw32 : Outport  Port=374
  VOUTP_5vAPS2PwrErrDTC_raw32 : Outport  Port=375
  VOUTP_EPBLockTODTC_raw32 : Outport  Port=376
  VOUTP_EPBUnlockTODTC_raw32 : Outport  Port=377
  VOUTP_LimpHomeActTmp_flg : Outport  Port=378
  VOUTP_DTCDetect_enum : Outport  Port=379
  VOUTP_EngagePFail_flg : Outport  Port=380
  VOUTP_DisengagePFail_flg : Outport  Port=381
  VOUTP_VCURAPSErrLv2_flg : Outport  Port=382
  VOUTP_VCURAPSErrLv3_flg : Outport  Port=383
  VOUTP_EDriveSysErrShifterErr_flg : Outport  Port=384
  VOUTP_LVSysErrPwrOutErr_flg : Outport  Port=385
  VOUTP_HVRlyOpFail_flg : Outport  Port=386
  VOUTP_MCUActDisFail_flg : Outport  Port=387
  VOUTP_VCUBrkSWSta_enum : Outport  Port=388
  VOUTP_VCUFLDoorSta_flg : Outport  Port=389
  VOUTP_VCUFRDoorSta_flg : Outport  Port=390
  VOUTP_VCURLDoorSta_flg : Outport  Port=391
  VOUTP_VCURRDoorSta_flg : Outport  Port=392
  VOUTP_SysAllowReadySta_flg : Outport  Port=393
  VOUTP_VCUHoodSWSta_flg : Outport  Port=394
  VOUTP_VCUTailgateSWSta_flg : Outport  Port=395
  VOUTP_ActAPSPosn_pct : Outport  Port=396
  VOUTP_EAPS1MIN_pct : Outport  Port=397
  VOUTP_EAPS2MIN_pct : Outport  Port=398
  VOUTP_ResetPedalZeroPosStart_flg : Outport  Port=399
  VOUTP_EAPS1NRM_pct : Outport  Port=400
  VOUTP_EAPS2NRM_pct : Outport  Port=401
  VOUTP_VSS_kph : Outport  Port=402
  VOUTP_RUNTM_s : Outport  Port=403
  VOUTP_MILDIST_km : Outport  Port=404
  VOUTP_WARMUPS_cnt : Outport  Port=405
  VOUTP_CLRDIST_km : Outport  Port=406
  VOUTP_APPD_pct : Outport  Port=407
  VOUTP_APPE_pct : Outport  Port=408
  VOUTP_MILTIME_min : Outport  Port=409
  VOUTP_CLRTIME_min : Outport  Port=410
  VOUTP_BATSOC_pct : Outport  Port=411
  VOUTP_HEVBATT_V : Outport  Port=412
  VOUTP_ODOMETER_km : Outport  Port=413
  VOUTP_BATSOH_pct : Outport  Port=414
  VOUTP_HVBCellVoltMin_V : Outport  Port=415
  VOUTP_HVBCellVoltMax_V : Outport  Port=416
  VOUTP_HVESSCHARGELIM_kW : Outport  Port=417
  VOUTP_HVESSCHARGEACT_kW : Outport  Port=418
  VOUTP_HVESSENER_Whps : Outport  Port=419
  VOUTP_NUMPSATRIPSFLTMEMCLR_cnt : Outport  Port=420
  VOUTP_HVBattCurr_Ahps : Outport  Port=421
  VOUTP_PSAR_sec : Outport  Port=422
  VOUTP_PSAL_sec : Outport  Port=423
  VOUTP_IPSAR_sec : Outport  Port=424
  VOUTP_IPSAL_sec : Outport  Port=425
  VOUTP_CPSAR_sec : Outport  Port=426
  VOUTP_CPSAL_sec : Outport  Port=427
  VOUTP_HVBNAH_Ahr : Outport  Port=428
  VOUTP_HVBNE_kWh : Outport  Port=429
  VOUTP_IGNCNTR_cnt : Outport  Port=430
  VOUTP_TNBCPSAR_Ahr : Outport  Port=431
  VOUTP_TNBCPSAL_Ahr : Outport  Port=432
  VOUTP_TNECPSAR_kWh : Outport  Port=433
  VOUTP_TNECPSAL_kWh : Outport  Port=434
  VOUTP_TEBPSAR_kWh : Outport  Port=435
  VOUTP_TEBPSAL_kWh : Outport  Port=436
  VOUTP_TGEOVCR_kWh : Outport  Port=437
  VOUTP_TGEOVCL_kWh : Outport  Port=438
  VOUTP_GECHGOVCDCR_kWh : Outport  Port=439
  VOUTP_GECHGOVCDCL_kWh : Outport  Port=440
  VOUTP_GECHGOVCACR_kWh : Outport  Port=441
  VOUTP_GECHGOVCACL_kWh : Outport  Port=442
  VOUTP_RESSV2XENNONPSAR_kWh : Outport  Port=443
  VOUTP_RESSV2XENNONPSAL_kWh : Outport  Port=444
  VOUTP_PKER_kphsqr : Outport  Port=445
  VOUTP_PKEL_kphsqr : Outport  Port=446
  VOUTP_ResetCDEODTR_km : Outport  Port=447
  VOUTP_CDEODTR_km : Outport  Port=448
  VOUTP_CDEODTL_km : Outport  Port=449
  VOUTP_AvgBattTempPSAR_C : Outport  Port=450
  VOUTP_AvgBattTempPSAL_C : Outport  Port=451
  VOUTP_AvgBattTempOVCR_C : Outport  Port=452
  VOUTP_AvgBattTempOVCL_C : Outport  Port=453
  VOUTP_AvgBattTempOFFR_C : Outport  Port=454
  VOUTP_AvgBattTempOFFL_C : Outport  Port=455
  VOUTP_QTYPSATRIPSR_cnt : Outport  Port=456
  VOUTP_QTYPSATRIPSL_cnt : Outport  Port=457
  VOUTP_RESSCNTDODRNGR_cnt : Outport  Port=458
  VOUTP_RESSCNTDODRNGL_cnt : Outport  Port=459
  VOUTP_ETMATOER_kWh : Outport  Port=460
  VOUTP_ETMATOEL_kWh : Outport  Port=461
  VOUTP_ETMBTOER_kWh : Outport  Port=462
  VOUTP_ETMBTOEL_kWh : Outport  Port=463
  VOUTP_RESSTIMESOCPSARNGR_s : Outport  Port=464
  VOUTP_RESSTIMESOCPSARNGL_s : Outport  Port=465
  VOUTP_RESSTIMESOCCHGRNGR_s : Outport  Port=466
  VOUTP_RESSTIMESOCCHGRNGL_s : Outport  Port=467
  VOUTP_RESSTIMESOCOFFRNGR_s : Outport  Port=468
  VOUTP_RESSTIMESOCOFFRNGL_s : Outport  Port=469
  VOUTP_MAXBATTEMPL_C : Outport  Port=470
  VOUTP_MINBATTEMPL_C : Outport  Port=471
  VOUTP_AVGBATTEMPL_C : Outport  Port=472
  VOUTP_PROTOCOLID_enum : Outport  Port=473
  VOUTP_RESSTTEMPRNGAXIS_enum : Outport  Port=474
  VOUTP_RESSTIMESOCRNGAXIS_enum : Outport  Port=475
  VOUTP_RESSCNTSDODRNGAXIS_enum : Outport  Port=476
  VOUTP_CALID_cnt : Outport  Port=477
  VOUTP_ECUNAME_cnt : Outport  Port=478
  VOUTP_PKERNumerator_kphsqr : Outport  Port=479
  VOUTP_PKELNumerator_kphsqr : Outport  Port=480
  VOUTP_BattTempPSAR_sec : Outport  Port=481
  VOUTP_BattTempPSAL_sec : Outport  Port=482
  VOUTP_OVCR_sec : Outport  Port=483
  VOUTP_OVCL_sec : Outport  Port=484
  VOUTP_OFFR_sec : Outport  Port=485
  VOUTP_OFFL_sec : Outport  Port=486
  VOUTP_AVGBATTEMPL_sec : Outport  Port=487
  VOUTP_VinCode_cnt : Outport  Port=488
  VOUTP_STASUP_enum : Outport  Port=489
  VOUTP_HEVMODE_enum : Outport  Port=490
  VOUTP_HVBATT_A : Outport  Port=491
  VOUTP_DIDModelVersion_raw : Outport  Port=492
  VOUTP_DIDModelVersionChksum_raw : Outport  Port=493
  VOUTP_DKCTimeSN_cnt : Outport  Port=494
  VOUTP_DKCAuthSta_enum : Outport  Port=495
  VOUTP_TimeSNDKCFbk_cnt : Outport  Port=496
  VOUTP_KeyMissSta_flg : Outport  Port=497
  VOUTP_KeyModeSta_enum : Outport  Port=498
  VOUTP_DkeyShowIVISta_enum : Outport  Port=499
  VOUTP_KeyAreaPS_enum : Outport  Port=500
  VOUTP_KeyAreaLockUnlock_enum : Outport  Port=501
  VOUTP_PCommandToBCM_enum : Outport  Port=502
  VOUTP_DKeyWelcomeSta_enum : Outport  Port=503
  VOUTP_KeyAreaPTG_enum : Outport  Port=504
  VOUTP_KeyAreaSPTGSta_enum : Outport  Port=505
  VOUTP_UIDLowPowerSta_enum : Outport  Port=506
  VOUTP_DkeyAreaRAPSSta_enum : Outport  Port=507
  VOUTP_ParkingModeCmd_enum : Outport  Port=508
  VOUTP_KeyNumSta_enum : Outport  Port=509
  VOUTP_KeyTypeSta_enum : Outport  Port=510
  VOUTP_FDCDKCAllowSleep_flg : Outport  Port=511
  VOUTP_JudgeKeepUnlockZone_flg : Outport  Port=512
  VOUTP_DISCTurn_flg : Outport  Port=513
  VOUTP_DISCTargetSpd_kph : Outport  Port=514
  VOUTP_DISCSta_enum : Outport  Port=515
  VOUTP_DISCButtSta_flg : Outport  Port=516
  VOUTP_AllCANTxReq_flg : Outport  Port=517
  VOUTP_NMmTxReq_flg : Outport  Port=518
  VOUTP_Awake_enum : Outport  Port=519
  VOUTP_CSB_flg : Outport  Port=520
  VOUTP_ErrorState_enum : Outport  Port=521
  VOUTP_NodeID_enum : Outport  Port=522
  VOUTP_PNI_flg : Outport  Port=523
  VOUTP_RptMsgReq_flg : Outport  Port=524
  VOUTP_WakeUp_enum : Outport  Port=525
  VOUTP_ActiveWU_flg : Outport  Port=526
  VOUTP_SysNMmSta_enum : Outport  Port=527
  VOUTP_NetworkReq_flg : Outport  Port=528
  VOUTP_SysPowerMode_enum : Outport  Port=529
  VOUTP_PowerUpState_enum : Outport  Port=530
  VOUTP_PowerDownState_enum : Outport  Port=531
  VOUTP_ChrgState_enum : Outport  Port=532
  VOUTP_PowerUpFault_enum : Outport  Port=533
  VOUTP_PowerDownFault_enum : Outport  Port=534
  VOUTP_ChrgFault_enum : Outport  Port=535
  VOUTP_IRCRlyClose_flg : Outport  Port=536
  VOUTP_IGNRlyClose_flg : Outport  Port=537
  VOUTP_BattHVDem_enum : Outport  Port=538
  VOUTP_DCDCRlyDem_enum : Outport  Port=539
  VOUTP_CACRlyDem_enum : Outport  Port=540
  VOUTP_MCUHVLoopDem_enum : Outport  Port=541
  VOUTP_EHPSRlyDem_enum : Outport  Port=542
  VOUTP_ACHVLoopDem_enum : Outport  Port=543
  VOUTP_HVSysReady_enum : Outport  Port=544
  VOUTP_DrivelineRelease_enum : Outport  Port=545
  VOUTP_ActiveDischargeReq_enum : Outport  Port=546
  VOUTP_VCUMCUEn_flg : Outport  Port=547
  VOUTP_VCUMCUFailRst_flg : Outport  Port=548
  VOUTP_HVILFail_flg : Outport  Port=549
  VOUTP_LostHVComActivePwrDown_flg : Outport  Port=550
  VOUTP_LVBattLowInd_enum : Outport  Port=551
  VOUTP_ChrgPowerUpFail_flg : Outport  Port=552
  VOUTP_ChrgBCUHVFail_flg : Outport  Port=553
  VOUTP_HVFailureChkPass_flg : Outport  Port=554
  VOUTP_HVILDetectFail_flg : Outport  Port=555
  VOUTP_V2BLifeSig_cnt : Outport  Port=556
  VOUTP_V2BAux1OnOff_enum : Outport  Port=557
  VOUTP_V2BAux2OnOff_enum : Outport  Port=558
  VOUTP_V2BAux3OnOff_enum : Outport  Port=559
  VOUTP_V2BMainPosRlySta_enum : Outport  Port=560
  VOUTP_V2BMainPosRlyFit_enum : Outport  Port=561
  VOUTP_V2BACPosRlySta_enum : Outport  Port=562
  VOUTP_V2BACPosRlyFit_enum : Outport  Port=563
  VOUTP_V2BAirPosRlySta_enum : Outport  Port=564
  VOUTP_V2BAirPosRlyFit_enum : Outport  Port=565
  VOUTP_V2BOilPosRlySta_enum : Outport  Port=566
  VOUTP_V2BOilPosRlyFit_enum : Outport  Port=567
  VOUTP_V2BDCDCPosRlySta_enum : Outport  Port=568
  VOUTP_V2BDCDCPosRlyFit_enum : Outport  Port=569
  VOUTP_V2BAux1RlySta_enum : Outport  Port=570
  VOUTP_V2BAux1RlyFit_enum : Outport  Port=571
  VOUTP_V2BAux2RlySta_enum : Outport  Port=572
  VOUTP_V2BAux2RlyFit_enum : Outport  Port=573
  VOUTP_V2BAux3RlySta_enum : Outport  Port=574
  VOUTP_V2BAux3RlyFit_enum : Outport  Port=575
  VOUTP_V2BAux4RlySta_enum : Outport  Port=576
  VOUTP_V2BAux4RlyFit_enum : Outport  Port=577
  VOUTP_VCULife1_cnt : Outport  Port=578
  VOUTP_VCULife2_cnt : Outport  Port=579
  VOUTP_VSPFunc_enum : Outport  Port=580
  VOUTP_VSPIGNKeySta_enum : Outport  Port=581
  VOUTP_VSPReversed_flg : Outport  Port=582
  VOUTP_VSPTurnRight_enum : Outport  Port=583
  VOUTP_VSPTurnLeft_enum : Outport  Port=584
  VOUTP_FogTMSRlyCMD_enum : Outport  Port=585
  VOUTP_DCCurr_A : Outport  Port=586
  VOUTP_DCVol_V : Outport  Port=587
  VOUTP_Keystatus_enum : Outport  Port=588
  VOUTP_EmergencyShutDown_flg : Outport  Port=589
  VOUTP_triggerBAM_flg : Outport  Port=590
  VOUTP_CFGEM1Ctrl_raw : Outport  Port=591
  VOUTP_CFGEM1BAMTSize_raw : Outport  Port=592
  VOUTP_CFGEM1BAMTNum_raw : Outport  Port=593
  VOUTP_CFGEM1BAMRsv_raw : Outport  Port=594
  VOUTP_CFGEM1BAMPGN_raw : Outport  Port=595
  VOUTP_triggerDT_flg : Outport  Port=596
  VOUTP_DTbyte0_raw : Outport  Port=597
  VOUTP_DTbyte1_raw : Outport  Port=598
  VOUTP_DTbyte2_raw : Outport  Port=599
  VOUTP_DTbyte3_raw : Outport  Port=600
  VOUTP_DTbyte4_raw : Outport  Port=601
  VOUTP_DTbyte5_raw : Outport  Port=602
  VOUTP_DTbyte6_raw : Outport  Port=603
  VOUTP_DTbyte7_raw : Outport  Port=604
  VOUTP_HWVer1_cnt : Outport  Port=605
  VOUTP_HWVer2_cnt : Outport  Port=606
  VOUTP_HWVer3_cnt : Outport  Port=607
  VOUTP_CarModel1_cnt : Outport  Port=608
  VOUTP_CarModel2_cnt : Outport  Port=609
  VOUTP_CarModel3_cnt : Outport  Port=610
  VOUTP_ECU1_cnt : Outport  Port=611
  VOUTP_ECU2_cnt : Outport  Port=612
  VOUTP_Major1_cnt : Outport  Port=613
  VOUTP_Major2_cnt : Outport  Port=614
  VOUTP_Minor1_cnt : Outport  Port=615
  VOUTP_Minor2_cnt : Outport  Port=616
  VOUTP_Patch1_cnt : Outport  Port=617
  VOUTP_Patch2_cnt : Outport  Port=618
  VOUTP_Country1_cnt : Outport  Port=619
  VOUTP_Country2_cnt : Outport  Port=620
  VOUTP_Variation_cnt : Outport  Port=621
  VOUTP_Dash1_cnt : Outport  Port=622
  VOUTP_Change1_cnt : Outport  Port=623
  VOUTP_Change2_cnt : Outport  Port=624
  VOUTP_Dash2_cnt : Outport  Port=625
  VOUTP_SHA1_cnt : Outport  Port=626
  VOUTP_SHA2_cnt : Outport  Port=627
  VOUTP_SHA3_cnt : Outport  Port=628
  VOUTP_SHA4_cnt : Outport  Port=629
  VOUTP_SHA5_cnt : Outport  Port=630
  VOUTP_SHA6_cnt : Outport  Port=631
  VOUTP_SHA7_cnt : Outport  Port=632
  VOUTP_SHA8_cnt : Outport  Port=633
  VOUTP_NvWriteReqRisingEdge_flg : Outport  Port=634
  VOUTP_FdcSlpReqRisingEdge_flg : Outport  Port=635
  VOUTP_FdcSlpTime_sec : Outport  Port=636
  VOUTP_PmicBootReason_enum : Outport  Port=637
  VOUTP_WisrBootReason_raw32 : Outport  Port=638
  VOUTP_AcoreRebootCmdACK_flg : Outport  Port=639
  VOUTP_CurrentNmState_enum : Outport  Port=640
  VOUTP_ECUGen1_cnt : Outport  Port=641
  VOUTP_ECUGen2_cnt : Outport  Port=642
  VOUTP_PmicBootPath_raw32 : Outport  Port=643
  VOUTP_DrivingMode_cnt : Outport  Port=644
  VOUTP_ModelYear_cnt : Outport  Port=645
  VOUTP_EWPPEReq_rpm : Outport  Port=646
  VOUTP_CoolFanReq_pct : Outport  Port=647
  VOUTP_AfterrunningMode_flg : Outport  Port=648
  VOUTP_LFBatWarn_flg : Outport  Port=649
  VOUTP_RFBatWarn_flg : Outport  Port=650
  VOUTP_LRBatWarn_flg : Outport  Port=651
  VOUTP_RRBatWarn_flg : Outport  Port=652
  VOUTP_LFWheelPress_raw8 : Outport  Port=653
  VOUTP_RFWheelPress_raw8 : Outport  Port=654
  VOUTP_LRWheelPress_raw8 : Outport  Port=655
  VOUTP_RRWheelPress_raw8 : Outport  Port=656
  VOUTP_LFWheelTemp_C : Outport  Port=657
  VOUTP_RFWheelTemp_C : Outport  Port=658
  VOUTP_LRWheelTemp_C : Outport  Port=659
  VOUTP_RRWheelTemp_C : Outport  Port=660
  VOUTP_LFSensorFail_flg : Outport  Port=661
  VOUTP_RFSensorFail_flg : Outport  Port=662
  VOUTP_LRSensorFail_flg : Outport  Port=663
  VOUTP_RRSensorFail_flg : Outport  Port=664
  VOUTP_LFWheelDebug_flg : Outport  Port=665
  VOUTP_LRWheelDebug_flg : Outport  Port=666
  VOUTP_RFWheelDebug_flg : Outport  Port=667
  VOUTP_RRWheelDebug_flg : Outport  Port=668
  VOUTP_TPMSResButtAllow_flg : Outport  Port=669
  VOUTP_TPMSCaliButtAllow_flg : Outport  Port=670
  VOUTP_LFPressIndi_enum : Outport  Port=671
  VOUTP_RFPressIndi_enum : Outport  Port=672
  VOUTP_LRPressIndi_enum : Outport  Port=673
  VOUTP_RRPressIndi_enum : Outport  Port=674
  VOUTP_TPMSWarnIndi_enum : Outport  Port=675
  VOUTP_LFWheelTmpIndi_flg : Outport  Port=676
  VOUTP_RFWheelTmpIndi_flg : Outport  Port=677
  VOUTP_LRWheelTmpIndi_flg : Outport  Port=678
  VOUTP_RRWheelTmpIndi_flg : Outport  Port=679
  VOUTP_LFWheelPSW_raw8 : Outport  Port=680
  VOUTP_LRWheelPSW_raw8 : Outport  Port=681
  VOUTP_RFWheelPSW_raw8 : Outport  Port=682
  VOUTP_RRWheelPSW_raw8 : Outport  Port=683
  VOUTP_CWheelTips_enum : Outport  Port=684
  VOUTP_AutoLTips_enum : Outport  Port=685
  VOUTP_LFSensorMode_flg : Outport  Port=686
  VOUTP_RFSensorMode_flg : Outport  Port=687
  VOUTP_LRSensorMode_flg : Outport  Port=688
  VOUTP_RRSensorMode_flg : Outport  Port=689
  VOUTP_S1ID_raw32 : Outport  Port=690
  VOUTP_S2ID_raw32 : Outport  Port=691
  VOUTP_S3ID_raw32 : Outport  Port=692
  VOUTP_S4ID_raw32 : Outport  Port=693
  VOUTP_S1L_enum : Outport  Port=694
  VOUTP_S2L_enum : Outport  Port=695
  VOUTP_S3L_enum : Outport  Port=696
  VOUTP_S4L_enum : Outport  Port=697
  VOUTP_ALFin_flg : Outport  Port=698
  VOUTP_LFP20_raw8 : Outport  Port=699
  VOUTP_RFP20_raw8 : Outport  Port=700
  VOUTP_LRP20_raw8 : Outport  Port=701
  VOUTP_RRP20_raw8 : Outport  Port=702
  VOUTP_FAT_flg : Outport  Port=703
  VOUTP_IDin_raw32 : Outport  Port=704
  VOUTP_S1WheelDebugALTU_pct : Outport  Port=705
  VOUTP_S2WheelDebugALTU_pct : Outport  Port=706
  VOUTP_S3WheelDebugALTU_pct : Outport  Port=707
  VOUTP_S4WheelDebugALTU_pct : Outport  Port=708
  VOUTP_ID1messageALTU_raw8 : Outport  Port=709
  VOUTP_ID2messageALTU_raw8 : Outport  Port=710
  VOUTP_ID3messageALTU_raw8 : Outport  Port=711
  VOUTP_ID4messageALTU_raw8 : Outport  Port=712
  VOUTP_Chkfin_flg : Outport  Port=713
  VOUTP_SetIDLoc_flg : Outport  Port=714
  VOUTP_TPMSStorge_flg : Outport  Port=715
  VOUTP_ChkStorge_flg : Outport  Port=716
  VOUTP_TPMSResButt_flg : Outport  Port=717
  VOUTP_LFPindi_enum : Outport  Port=718
  VOUTP_RFPind_enum : Outport  Port=719
  VOUTP_LRPindi_enum : Outport  Port=720
  VOUTP_RRPindi_enum : Outport  Port=721
  VOUTP_WriteChkLFID_raw : Outport  Port=722
  VOUTP_WriteChkRFID_raw : Outport  Port=723
  VOUTP_WriteChkLRID_raw : Outport  Port=724
  VOUTP_WriteChkRRID_raw : Outport  Port=725
  VOUTP_WriteChkfinLFID_raw : Outport  Port=726
  VOUTP_WriteChkfinRFID_raw : Outport  Port=727
  VOUTP_WriteChkfinLRID_raw : Outport  Port=728
  VOUTP_WriteChkfinRRID_raw : Outport  Port=729
  VOUTP_Flashchkdatavalid_enum : Outport  Port=730
  VOUTP_Flashdatavalid_enum : Outport  Port=731
  VOUTP_unlearnSfali_flg : Outport  Port=732
  VOUTP_unlearnSfailvalid_enum : Outport  Port=733
  VOUTP_Prepresstempvalid_enum : Outport  Port=734
  VOUTP_FlashS1ID_raw : Outport  Port=735
  VOUTP_FlashS2ID_raw : Outport  Port=736
  VOUTP_FlashS3ID_raw : Outport  Port=737
  VOUTP_FlashS4ID_raw : Outport  Port=738
  VOUTP_FlashIDvalid_enum : Outport  Port=739
  VOUTP_WritingCnt_enum : Outport  Port=740
  VOUTP_TPMSTLCmd_flg : Outport  Port=741
  VOUTP_LProgress_enum : Outport  Port=742
  VOUTP_TPMSSensorIDRegStart_flg : Outport  Port=743
  VOUTP_ModelVersion_raw : Outport  Port=744
  VOUTP_ModelVersionChksum_raw : Outport  Port=745
  VOUTP_VCUMCUCtrlMdTQD_enum : Outport  Port=746
  VOUTP_CreepSpdReq_rpm : Outport  Port=747
  VOUTP_CreepIND_enum : Outport  Port=748
  VOUTP_ActTUpAIND_enum : Outport  Port=749
  VOUTP_VCUMCUDemHiPosVal_rpm : Outport  Port=750
  VOUTP_VehAcclLimitTG_mps2 : Outport  Port=751
  VOUTP_VCUEBSHHSw_enum : Outport  Port=752
  VOUTP_VCUEBSRd4BR_enum : Outport  Port=753
  VOUTP_ParkingProtectWarning_flg : Outport  Port=754
  VOUTP_ActDriveMode_enum : Outport  Port=755
  VOUTP_VCU4PweLmtInd_flg : Outport  Port=756
  VOUTP_GearFlashIndDis_flg : Outport  Port=757
  VOUTP_GearFlashInd_flg : Outport  Port=758
  VOUTP_SpdLimSta_flg : Outport  Port=759
  VOUTP_VehSpdLimitTG_kph : Outport  Port=760
  VOUTP_VCUTMVehSpd_kph : Outport  Port=761
  VOUTP_TMTqReq_Nm : Outport  Port=762
  VOUTP_VCUBCMBuzzReq_flg : Outport  Port=763
  VOUTP_VCUEBSHBSw_enum : Outport  Port=764
  VOUTP_EVCU1ActDrvMode_enum : Outport  Port=765
  VOUTP_EVCU1WheelSlipdet_enum : Outport  Port=766
  VOUTP_EVCU1EMotorSpd_rpm : Outport  Port=767
  VOUTP_EVCU1EMotorOvrerSpd_enum : Outport  Port=768
  VOUTP_EVCU1EMotorPerformance_pct : Outport  Port=769
  VOUTP_EVCU1EBrakeTorqLow_enum : Outport  Port=770
  VOUTP_EVCU2MaxTorqAvail_pct : Outport  Port=771
  VOUTP_EVCU2MinTorqAvail_pct : Outport  Port=772
  VOUTP_EEC3NFricPercTorq_pct : Outport  Port=773
  VOUTP_EEC3EMPressLoss_pct : Outport  Port=774
  VOUTP_ETC2ActDriveDirect_enum : Outport  Port=775
  VOUTP_RC1PctTrqP4_pct : Outport  Port=776
  VOUTP_RC1PctTrqPekTrqP5_pct : Outport  Port=777
  VOUTP_EMRC1EMTquModeDrvBrk_enum : Outport  Port=778
  VOUTP_EMRC1ActEMpTrq_pct : Outport  Port=779
  VOUTP_EMRC1ActEMOutSftSpd_rpm : Outport  Port=780
  VOUTP_EMRC1ActEMpTrqHrls_pct : Outport  Port=781
  VOUTP_EMRC1ActMaxAvaEMRecpTrq_pct : Outport  Port=782
  VOUTP_EC1EMSpdIdleP1_rpm : Outport  Port=783
  VOUTP_EC1PercTorqIdleP1_pct : Outport  Port=784
  VOUTP_EC1EMSpdIdleP2_rpm : Outport  Port=785
  VOUTP_EC1PercTorqIdleP2_pct : Outport  Port=786
  VOUTP_EC1EMSpdIdleP3_rpm : Outport  Port=787
  VOUTP_EC1PercTorqIdleP3_pct : Outport  Port=788
  VOUTP_EC1EMSpdIdleP4_rpm : Outport  Port=789
  VOUTP_EC1PercTorqIdleP4_pct : Outport  Port=790
  VOUTP_EC1PercTorqIdleP5_pct : Outport  Port=791
  VOUTP_EC1EMSpdIdleP5_rpm : Outport  Port=792
  VOUTP_EC1EMRefTorq_Nm : Outport  Port=793
  VOUTP_EC1EMMaxMEngOvrSP7_rpm : Outport  Port=794
  VOUTP_EC1EMMaxMOvrTmt_s : Outport  Port=795
  VOUTP_EC1EMReqSpdCtrlLoLmt_rpm : Outport  Port=796
  VOUTP_EC1EMReqTrqCtrlLoLmt_pct : Outport  Port=797
  VOUTP_EC1EMReqSpdCtrlUpLmt_rpm : Outport  Port=798
  VOUTP_EC1EMReqTrqCtrlUpLmt_pct : Outport  Port=799
  VOUTP_EC1EMExtRSCtrlUpLmt_rpm : Outport  Port=800
  VOUTP_EC1EMMomOfInertia_kgpm2 : Outport  Port=801
  VOUTP_EC1EMDefTrqLmt_rpm : Outport  Port=802
  VOUTP_EC1EMSupVarRTSC1MSG_cnt : Outport  Port=803
  VOUTP_EC1EMSupTSC1CtrlPG1_cnt : Outport  Port=804
  VOUTP_EC1EMSupTSC1CtrlPG3_cnt : Outport  Port=805
  VOUTP_EC1EMSupTSC1CtrlPG2_cnt : Outport  Port=806
  VOUTP_EC1EMSupTSC1CtrlPG4_cnt : Outport  Port=807
  VOUTP_EC1EMSpdHdleP6_rpm : Outport  Port=808
  VOUTP_EC1EMGainEndSpdGvn_gain : Outport  Port=809
  VOUTP_RC1RetType_enum : Outport  Port=810
  VOUTP_RC1RetLocat_enum : Outport  Port=811
  VOUTP_RC1RetCtrlMth_enum : Outport  Port=812
  VOUTP_RC1RetSpdIdleP1_rpm : Outport  Port=813
  VOUTP_RC1PctTrqIdleP1_pct : Outport  Port=814
  VOUTP_RC1MaxRetSpdP2_rpm : Outport  Port=815
  VOUTP_RC1RetSpdP2_pct : Outport  Port=816
  VOUTP_RC1MaxRetSpdP3_rpm : Outport  Port=817
  VOUTP_RC1PctTrqP3_pct : Outport  Port=818
  VOUTP_RC1RefRetTrq_Nm : Outport  Port=819
  VOUTP_RC1RetSpdPekTrqP5_Nm : Outport  Port=820
  VOUTP_RC1RetSpdP4_rpm : Outport  Port=821
  VOUTP_VCUMCUDemLoNegVal_rpm : Outport  Port=822
  VOUTP_VCUMCUDemSpd_rpm : Outport  Port=823
  VOUTP_VCUMCUGearSta_enum : Outport  Port=824
  VOUTP_TUpAIND_enum : Outport  Port=825
  VOUTP_ETC1ShiftrPgs_enum : Outport  Port=826
  VOUTP_EVCU1RecuperHighSta_enum : Outport  Port=827
  VOUTP_EMRC1DrvDemEMRtapTrq_pct : Outport  Port=828
  VOUTP_EMRC1RetSelNonEng_pct : Outport  Port=829
  VOUTP_EMRC1SACtrlDev_cnt : Outport  Port=830
  VOUTP_VCUMCUHandBrk_flg : Outport  Port=831
  VOUTP_VCUMCUFootBrk_flg : Outport  Port=832
  VOUTP_FrTMTqReq_Nm : Outport  Port=833
  VOUTP_RrTMTqReq_Nm : Outport  Port=834
  VOUTP_ReqOBCV2LEna_enum : Outport  Port=835
  VOUTP_ReqV2LIVIPopup_enum : Outport  Port=836
  VOUTP_ReqV2LIVIDisChrg_enum : Outport  Port=837
  VOUTP_ReqOBCExtrV2LEna_enum : Outport  Port=838
  VOUTP_ReqOBCIntrV2LEna_enum : Outport  Port=839
  VOUTP_HVPO120VGrpALDSt_enum : Outport  Port=840
  VOUTP_HVPO120VGrpBLDSt_enum : Outport  Port=841
  VOUTP_FeatSetSpdFinal_raw32 : Outport  Port=842
  VOUTP_VehicleSpeed_mph : Outport  Port=843
  VOUTP_VehicleSpeed_kph : Outport  Port=844
  VOUTP_MeterIndSpeed_raw32 : Outport  Port=845
  VOUTP_VMCAEBCtrlAvail_flg : Outport  Port=846
  VOUTP_VMCACCCtrlAvail_flg : Outport  Port=847
  VOUTP_VMCCCCtrlAvail_flg : Outport  Port=848
  VOUTP_VMCMSACtrlAvail_flg : Outport  Port=849
  VOUTP_FeatArbitrSta_enum : Outport  Port=850
  VOUTP_FeatReqSpd_kph : Outport  Port=851
  VOUTP_JerkPCT_pct : Outport  Port=852
  VOUTP_LimitPCT_pct : Outport  Port=853
  VOUTP_FrontRearSlipRatioCtrl_flg : Outport  Port=854
  VOUTP_RearWhlSlipRatioCtrl_flg : Outport  Port=855
  VOUTP_SingleWhlSlipRatioCtrl_flg : Outport  Port=856
  VOUTP_LatAccCtrl_flg : Outport  Port=857
  VOUTP_SafetyCtrl_flg : Outport  Port=858
  VOUTP_SPD2ACCAct_flg : Outport  Port=859
  VOUTP_AccCalcuPID_mps2 : Outport  Port=860
  VOUTP_ISOAccLimit_mps2 : Outport  Port=861
  VOUTP_ISODecLimit_mps2 : Outport  Port=862
  VOUTP_ISOJerkLimit_mps3 : Outport  Port=863
  VOUTP_ACCRequiredAccel_mps2 : Outport  Port=864
  VOUTP_DISCReqAcc_mps2 : Outport  Port=865
  VOUTP_FeatArbitrFinal_enum : Outport  Port=866
  VOUTP_ActACCRequiredAccel_mps2 : Outport  Port=867
  VOUTP_LateralCtrl_flg : Outport  Port=868
  VOUTP_ADASLKASta_enum : Outport  Port=869
  VOUTP_LKAStrToqReq_Nm : Outport  Port=870
  VOUTP_LKATOIFault_flg : Outport  Port=871
  VOUTP_LKATOIAct_enum : Outport  Port=872
  VOUTP_ADASAEBReq_enum : Outport  Port=873
  VOUTP_ADASFaultSta_flg : Outport  Port=874
  VOUTP_AEBVehHoldReq_flg : Outport  Port=875
  VOUTP_ACCVehHoldReq_flg : Outport  Port=876
  VOUTP_ADASDBSReq_enum : Outport  Port=877
  VOUTP_ADASACCSta_enum : Outport  Port=878
  VOUTP_ACCObjDist_m : Outport  Port=879
  VOUTP_ACCObjRelSpd_mps : Outport  Port=880
  VOUTP_TimeGapLevel_enum : Outport  Port=881
  VOUTP_ACCJerkUpperLimit_mps3 : Outport  Port=882
  VOUTP_ACCComfortBandUpper_mps2 : Outport  Port=883
  VOUTP_ACCJerkLowerLimit_mps3 : Outport  Port=884
  VOUTP_ACCComfortBandLower_mps2 : Outport  Port=885
  VOUTP_ADASVehSpdLim_raw32 : Outport  Port=886
  VOUTP_ADASShftPosnReqA_flg : Outport  Port=887
  VOUTP_ADASShftPosnReq_enum : Outport  Port=888
  VOUTP_ADASForceIdle_flg : Outport  Port=889
  VOUTP_HazardWarningReq_flg : Outport  Port=890
  VOUTP_RightTurnLightReq_flg : Outport  Port=891
  VOUTP_LeftTurnLightReq_flg : Outport  Port=892
  VOUTP_ADASFCWSta_enum : Outport  Port=893
  VOUTP_ADASLDWSta_enum : Outport  Port=894
  VOUTP_ADASFltWrnReq_flg : Outport  Port=895
  VOUTP_ACCObjDstLvl_enum : Outport  Port=896
  VOUTP_ForceLowBeam_enum : Outport  Port=897
  VOUTP_ACCTakeoverReq_flg : Outport  Port=898
  VOUTP_ADASWarningMsg_enum : Outport  Port=899
  VOUTP_ADASCAMSpdLim_enum : Outport  Port=900
  VOUTP_TargetType_enum : Outport  Port=901
  VOUTP_ADASSLIFSpdLim_enum : Outport  Port=902
  VOUTP_LKAHODDisplayWarning_flg : Outport  Port=903
  VOUTP_LKAHODSoundWarning_flg : Outport  Port=904
  VOUTP_ADASLFCSta_enum : Outport  Port=905
  VOUTP_ADASLaneModeL_enum : Outport  Port=906
  VOUTP_ADASLaneModeR_enum : Outport  Port=907
  VOUTP_ADASSLIFSta_enum : Outport  Port=908
  VOUTP_ADASISASta_enum : Outport  Port=909
  VOUTP_ADASLDWMute_flg : Outport  Port=910
  VOUTP_ADASFCWMute_flg : Outport  Port=911
  VOUTP_ADASLFCHandsOffWarning_enum : Outport  Port=912
  VOUTP_LVDADisabled_flg : Outport  Port=913
  VOUTP_LVDAMuteSta_enum : Outport  Port=914
  VOUTP_LVDAFailinfo_flg : Outport  Port=915
  VOUTP_LVDAWarning_flg : Outport  Port=916
  VOUTP_LVDAACCStatusInformation_flg : Outport  Port=917
  VOUTP_ADASLFCWarnSound_enum : Outport  Port=918
  VOUTP_FCMACCmode_enum : Outport  Port=919
  VOUTP_ADASLanetypeR_enum : Outport  Port=920
  VOUTP_ADASLanetypeL_enum : Outport  Port=921
  VOUTP_ADASLanecurveL_raw32 : Outport  Port=922
  VOUTP_ADASLanecurveR_raw32 : Outport  Port=923
  VOUTP_ADASAEBSta_enum : Outport  Port=924
  VOUTP_FCMLDWRequest_enum : Outport  Port=925
  VOUTP_FCMLDWFault_flg : Outport  Port=926
  VOUTP_ACCCtrlAvail_flg : Outport  Port=927
  VOUTP_ACCPedalOvrd_flg : Outport  Port=928
  VOUTP_TimeGapCalcu_s : Outport  Port=929
  VOUTP_CCCtrlSta_enum : Outport  Port=930
  VOUTP_MSACtrlSta_enum : Outport  Port=931
  VOUTP_APSCtrlAvail_flg : Outport  Port=932
  VOUTP_APSActive_flg : Outport  Port=933
  VOUTP_APSStaSys_enum : Outport  Port=934
  VOUTP_APSDecReqA_flg : Outport  Port=935
  VOUTP_APSDecReq_mps2 : Outport  Port=936
  VOUTP_APSReq_enum : Outport  Port=937
  VOUTP_LongAcc_Gps : Outport  Port=938
  VOUTP_CCMSASpdWar_flg : Outport  Port=939
  VOUTP_IMUEnaCmd_flg : Outport  Port=940
  VOUTP_CAASCtrlAvail_flg : Outport  Port=941
  VOUTP_CAASActive_flg : Outport  Port=942
  VOUTP_ExtraMSACtrlSta_enum : Outport  Port=943
  VOUTP_CalibratedAccX_G : Outport  Port=944
  VOUTP_CalibratedAccY_G : Outport  Port=945
  VOUTP_CalibratedAccZ_G : Outport  Port=946
  VOUTP_CalibratedGyroX_Dps : Outport  Port=947
  VOUTP_CalibratedGyroY_Dps : Outport  Port=948
  VOUTP_CalibratedGyroZ_Dps : Outport  Port=949
  VOUTP_FDCVMCAPSVRqEPSCtrl_flg : Outport  Port=950
  VOUTP_FDCVMCAPSAngleTarget_deg : Outport  Port=951
  VOUTP_FDCVMCAPSRqEPSCtrl_flg : Outport  Port=952
  VOUTP_FDCVMCAngCtrlTqWtGn_pct : Outport  Port=953
  VOUTP_FDCVMCDrInpTqBstAct_flg : Outport  Port=954
  VOUTP_FDCVMCMaxAngCtrlOutTqLim_Nm : Outport  Port=955
  VOUTP_FDCVMCDrInpTqBstGn_pct : Outport  Port=956
  wires:
  VACC_EACEnDemand_enum/1 -> VACC_EACEnDemand_enum_Inproc/1  "VACC_EACEnDemand_enum"
  VACC_EACEnDemand_enum_Inproc/1 -> UnitConverter1/1
  UnitConverter1/1 -> VOUTP_EACEnDemand_enum/1  "VOUTP_EACEnDemand_enum"
  VACC_CACTempOverHigh_flg/1 -> VACC_CACTempOverHigh_flg_Inproc/1  "VACC_CACTempOverHigh_flg"
  VACC_CACTempOverHigh_flg_Inproc/1 -> UnitConverter2/1
  UnitConverter2/1 -> VOUTP_CACTempOverHigh_flg/1  "VOUTP_CACTempOverHigh_flg"
  VACC_CACPresWarn_flg/1 -> VACC_CACPresWarn_flg_Inproc/1  "VACC_CACPresWarn_flg"
  VACC_CACPresWarn_flg_Inproc/1 -> UnitConverter3/1
  UnitConverter3/1 -> VOUTP_CACPresWarn_flg/1  "VOUTP_CACPresWarn_flg"
  VACC_CACPresReady_flg/1 -> VACC_CACPresReady_flg_Inproc/1  "VACC_CACPresReady_flg"
  VACC_CACPresReady_flg_Inproc/1 -> UnitConverter4/1
  UnitConverter4/1 -> VOUTP_CACPresReady_flg/1  "VOUTP_CACPresReady_flg"
  VACC_EHPSEnDemand_enum/1 -> VACC_EHPSEnDemand_enum_Inproc/1  "VACC_EHPSEnDemand_enum"
  VACC_EHPSEnDemand_enum_Inproc/1 -> UnitConverter5/1
  UnitConverter5/1 -> VOUTP_EHPSEnDemand_enum/1  "VOUTP_EHPSEnDemand_enum"
  VACC_CACOverrun_flg/1 -> VACC_CACOverrun_flg_Inproc/1  "VACC_CACOverrun_flg"
  VACC_CACOverrun_flg_Inproc/1 -> UnitConverter6/1
  UnitConverter6/1 -> VOUTP_CACOverrun_flg/1  "VOUTP_CACOverrun_flg"
  VACC_CACRunFail_flg/1 -> VACC_CACRunFail_flg_Inproc/1  "VACC_CACRunFail_flg"
  VACC_CACRunFail_flg_Inproc/1 -> UnitConverter7/1
  UnitConverter7/1 -> VOUTP_CACRunFail_flg/1  "VOUTP_CACRunFail_flg"
  VACC_CACFanReq_flg/1 -> VACC_CACFanReq_flg_Inproc/1  "VACC_CACFanReq_flg"
  VACC_CACFanReq_flg_Inproc/1 -> UnitConverter8/1
  UnitConverter8/1 -> VOUTP_CACFanReq_flg/1  "VOUTP_CACFanReq_flg"
  VACC_EHPSMotorDemSpd_rpm/1 -> VACC_EHPSMotorDemSpd_rpm_Inproc/1  "VACC_EHPSMotorDemSpd_rpm"
  VACC_EHPSMotorDemSpd_rpm_Inproc/1 -> UnitConverter9/1
  UnitConverter9/1 -> VOUTP_EHPSMotorDemSpd_rpm/1  "VOUTP_EHPSMotorDemSpd_rpm"
  VACC_EHPSSpdDemTimeout_flg/1 -> VACC_EHPSSpdDemTimeout_flg_Inproc/1  "VACC_EHPSSpdDemTimeout_flg"
  VACC_EHPSSpdDemTimeout_flg_Inproc/1 -> UnitConverter10/1
  UnitConverter10/1 -> VOUTP_EHPSSpdDemTimeout_flg/1  "VOUTP_EHPSSpdDemTimeout_flg"
  VACC_EHPSEnTimeout_flg/1 -> VACC_EHPSEnTimeout_flg_Inproc/1  "VACC_EHPSEnTimeout_flg"
  VACC_EHPSEnTimeout_flg_Inproc/1 -> UnitConverter11/1
  UnitConverter11/1 -> VOUTP_EHPSEnTimeout_flg/1  "VOUTP_EHPSEnTimeout_flg"
  VACC_EHPSDisEnTimeout_flg/1 -> VACC_EHPSDisEnTimeout_flg_Inproc/1  "VACC_EHPSDisEnTimeout_flg"
  VACC_EHPSDisEnTimeout_flg_Inproc/1 -> UnitConverter12/1
  UnitConverter12/1 -> VOUTP_EHPSDisEnTimeout_flg/1  "VOUTP_EHPSDisEnTimeout_flg"
  VACC_DCDCEnDemamd_enum/1 -> VACC_DCDCEnDemamd_enum_Inproc/1  "VACC_DCDCEnDemamd_enum"
  VACC_DCDCEnDemamd_enum_Inproc/1 -> UnitConverter13/1
  UnitConverter13/1 -> VOUTP_DCDCEnDemamd_enum/1  "VOUTP_DCDCEnDemamd_enum"
  VACC_EHPSSpdCtrlMode_enum/1 -> VACC_EHPSSpdCtrlMode_enum_Inproc/1  "VACC_EHPSSpdCtrlMode_enum"
  VACC_EHPSSpdCtrlMode_enum_Inproc/1 -> UnitConverter14/1
  UnitConverter14/1 -> VOUTP_EHPSSpdCtrlMode_enum/1  "VOUTP_EHPSSpdCtrlMode_enum"
  VACC_EACSpdDemand_rpm/1 -> VACC_EACSpdDemand_rpm_Inproc/1  "VACC_EACSpdDemand_rpm"
  VACC_EACSpdDemand_rpm_Inproc/1 -> UnitConverter15/1
  UnitConverter15/1 -> VOUTP_EACSpdDemand_rpm/1  "VOUTP_EACSpdDemand_rpm"
  VAPM_VehSpeed_kph/1 -> VAPM_VehSpeed_kph_Inproc/1  "VAPM_VehSpeed_kph"
  VAPM_VehSpeed_kph_Inproc/1 -> UnitConverter16/1
  UnitConverter16/1 -> VOUTP_VehSpeed_kph/1  "VOUTP_VehSpeed_kph"
  VAPM_VehSpeedTimeOut_flg/1 -> VAPM_VehSpeedTimeOut_flg_Inproc/1  "VAPM_VehSpeedTimeOut_flg"
  VAPM_VehSpeedTimeOut_flg_Inproc/1 -> UnitConverter17/1
  UnitConverter17/1 -> VOUTP_VehSpeedTimeOut_flg/1  "VOUTP_VehSpeedTimeOut_flg"
  VAPM_FSOffSw_enum/1 -> VAPM_FSOffSw_enum_Inproc/1  "VAPM_FSOffSw_enum"
  VAPM_FSOffSw_enum_Inproc/1 -> UnitConverter18/1
  UnitConverter18/1 -> VOUTP_FSOffSw_enum/1  "VOUTP_FSOffSw_enum"
  VAPM_FSOffSwTimeOut_flg/1 -> VAPM_FSOffSwTimeOut_flg_Inproc/1  "VAPM_FSOffSwTimeOut_flg"
  VAPM_FSOffSwTimeOut_flg_Inproc/1 -> UnitConverter19/1
  UnitConverter19/1 -> VOUTP_FSOffSwTimeOut_flg/1  "VOUTP_FSOffSwTimeOut_flg"
  VAPM_ChrgPlugSta_enum/1 -> VAPM_ChrgPlugSta_enum_Inproc/1  "VAPM_ChrgPlugSta_enum"
  VAPM_ChrgPlugSta_enum_Inproc/1 -> UnitConverter20/1
  UnitConverter20/1 -> VOUTP_ChrgPlugSta_enum/1  "VOUTP_ChrgPlugSta_enum"
  VAPM_PASDRMR_cm/1 -> VAPM_PASDRMR_cm_Inproc/1  "VAPM_PASDRMR_cm"
  VAPM_PASDRMR_cm_Inproc/1 -> UnitConverter21/1
  UnitConverter21/1 -> VOUTP_PASDRMR_cm/1  "VOUTP_PASDRMR_cm"
